simulink model "model"  (R2014a)
(part 5 of 6)

  _CN_240522248_230000_CN_261953891_230000/RConn1 -- T_261953891__/LConn1 -- _CN_261953891_230000_CN_262122922_230000/RConn1
  _CN_240522248_230000_CN_261953891_230000/RConn2 -- T_261953891__/LConn2 -- _CN_261953891_230000_CN_262122922_230000/RConn2
  _CN_240522248_230000_CN_261953891_230000/RConn3 -- T_261953891__/LConn3 -- _CN_261953891_230000_CN_262122922_230000/RConn3 -- bus92/LConn1
  T_204336141__/LConn1 -- _CN_204336141_230000_CN_194446718_230000/LConn1
  T_204336141__/LConn2 -- _CN_204336141_230000_CN_194446718_230000/LConn2
  _CN_204336141_230000_CN_194446718_230000/LConn3 -- T_204336141__/LConn3 -- bus93/LConn1
  T_194446718__Santa_Maria_3/LConn1 -- _CN_204336141_230000_CN_194446718_230000/RConn1
  T_194446718__Santa_Maria_3/LConn2 -- _CN_204336141_230000_CN_194446718_230000/RConn2
  _CN_204336141_230000_CN_194446718_230000/RConn3 -- T_194446718__Santa_Maria_3/LConn3 -- bus94/LConn1
  _CN_146723856_230000_CN_105353506_230000/LConn1 -- T_146723856_230000_Subestação_Maringá/LConn1 -- _CN_146723856_230000_CN_206109551_230000/LConn1 -- _CN_146723856_230000_CN_394083271_230000/LConn1
  _CN_146723856_230000_CN_105353506_230000/LConn2 -- T_146723856_230000_Subestação_Maringá/LConn2 -- _CN_146723856_230000_CN_206109551_230000/LConn2 -- _CN_146723856_230000_CN_394083271_230000/LConn2
  _CN_146723856_230000_CN_105353506_230000/LConn3 -- T_146723856_230000_Subestação_Maringá/LConn3 -- _CN_146723856_230000_CN_206109551_230000/LConn3 -- _CN_146723856_230000_CN_394083271_230000/LConn3 -- bus95/LConn1
  _CN_146723856_230000_CN_105353506_230000/RConn1 -- T_105353506_230000_Subestação_Apucarana/LConn1 -- Linha_de_Transmissão_CM_AP_CN_105353506_230000_CN_394083271_230000/LConn1 -- _CN_131689631_230000_CN_105353506_230000/LConn1 -- _CN_105361984_230000_CN_105353506_230000/LConn1
  _CN_146723856_230000_CN_105353506_230000/RConn2 -- T_105353506_230000_Subestação_Apucarana/LConn2 -- Linha_de_Transmissão_CM_AP_CN_105353506_230000_CN_394083271_230000/LConn2 -- _CN_131689631_230000_CN_105353506_230000/LConn2 -- _CN_105361984_230000_CN_105353506_230000/LConn2
  _CN_146723856_230000_CN_105353506_230000/RConn3 -- T_105353506_230000_Subestação_Apucarana/LConn3 -- Linha_de_Transmissão_CM_AP_CN_105353506_230000_CN_394083271_230000/LConn3 -- bus96/LConn1 -- _CN_131689631_230000_CN_105353506_230000/LConn3 -- _CN_105361984_230000_CN_105353506_230000/LConn3
  T_206109551_230000_Subestação_Sarandi/LConn1 -- _CN_146723856_230000_CN_206109551_230000/RConn1
  T_206109551_230000_Subestação_Sarandi/LConn2 -- _CN_146723856_230000_CN_206109551_230000/RConn2
  _CN_146723856_230000_CN_206109551_230000/RConn3 -- T_206109551_230000_Subestação_Sarandi/LConn3 -- bus97/LConn1
  _CN_146723856_230000_CN_394083271_230000/RConn1 -- T_394083271_230000;13800_Subestação_Campo_Mourão/LConn1 -- Linha_de_Transmissão_CM_AP_CN_105353506_230000_CN_394083271_230000/RConn1
  _CN_146723856_230000_CN_394083271_230000/RConn2 -- T_394083271_230000;13800_Subestação_Campo_Mourão/LConn2 -- Linha_de_Transmissão_CM_AP_CN_105353506_230000_CN_394083271_230000/RConn2
  _CN_146723856_230000_CN_394083271_230000/RConn3 -- T_394083271_230000;13800_Subestação_Campo_Mourão/LConn3 -- Linha_de_Transmissão_CM_AP_CN_105353506_230000_CN_394083271_230000/RConn3 -- bus98/LConn1
  _CN_323557394_230000_CN_303915320_230000/LConn1 -- T_323557394__/RConn1 -- L_323557394/LConn1
  _CN_323557394_230000_CN_303915320_230000/LConn2 -- T_323557394__/RConn2 -- L_323557394/LConn2
  _CN_323557394_230000_CN_303915320_230000/LConn3 -- T_323557394__/RConn3 -- L_323557394/LConn3 -- bus99/LConn1
  T_303915320__/LConn1 -- _CN_323557394_230000_CN_303915320_230000/RConn1
  T_303915320__/LConn2 -- _CN_323557394_230000_CN_303915320_230000/RConn2
  _CN_323557394_230000_CN_303915320_230000/RConn3 -- T_303915320__/LConn3 -- bus100/LConn1
  _CN_262826007_230000_CN_262826015_230000/LConn1 -- T_262826007__/RConn1 -- L_262826007/LConn1
  _CN_262826007_230000_CN_262826015_230000/LConn2 -- T_262826007__/RConn2 -- L_262826007/LConn2
  _CN_262826007_230000_CN_262826015_230000/LConn3 -- T_262826007__/RConn3 -- L_262826007/LConn3 -- bus101/LConn1
  T_262826015__/LConn1 -- _CN_262826007_230000_CN_262826015_230000/RConn1
  T_262826015__/LConn2 -- _CN_262826007_230000_CN_262826015_230000/RConn2
  _CN_262826007_230000_CN_262826015_230000/RConn3 -- T_262826015__/LConn3 -- bus102/LConn1
  _CN_241914909_230000_CN_241914913_230000/LConn1 -- T_241914909__/LConn1 -- _CN_241914909_230000_CN_241914935_230000/LConn1 -- _CN_241914909_230000_CN_242506367_230000/LConn1 -- _CN_241914909_230000_CN_242506209_230000/LConn1
  _CN_241914909_230000_CN_241914913_230000/LConn2 -- T_241914909__/LConn2 -- _CN_241914909_230000_CN_241914935_230000/LConn2 -- _CN_241914909_230000_CN_242506367_230000/LConn2 -- _CN_241914909_230000_CN_242506209_230000/LConn2
  _CN_241914909_230000_CN_241914913_230000/LConn3 -- T_241914909__/LConn3 -- _CN_241914909_230000_CN_241914935_230000/LConn3 -- _CN_241914909_230000_CN_242506367_230000/LConn3 -- bus103/LConn1 -- _CN_241914909_230000_CN_242506209_230000/LConn3
  _CN_241914909_230000_CN_241914913_230000/RConn1 -- T_241914913__/RConn1 -- L_241914913/LConn1
  _CN_241914909_230000_CN_241914913_230000/RConn2 -- T_241914913__/RConn2 -- L_241914913/LConn2
  _CN_241914909_230000_CN_241914913_230000/RConn3 -- T_241914913__/RConn3 -- L_241914913/LConn3 -- bus104/LConn1
  T_242506209__/LConn1 -- _CN_241914909_230000_CN_242506209_230000/RConn1
  T_242506209__/LConn2 -- _CN_241914909_230000_CN_242506209_230000/RConn2
  _CN_241914909_230000_CN_242506209_230000/RConn3 -- T_242506209__/LConn3 -- bus105/LConn1
  T_241914935__/LConn1 -- _CN_241914909_230000_CN_241914935_230000/RConn1
  T_241914935__/LConn2 -- _CN_241914909_230000_CN_241914935_230000/RConn2
  _CN_241914909_230000_CN_241914935_230000/RConn3 -- T_241914935__/LConn3 -- bus106/LConn1
  T_242506367__/LConn1 -- _CN_241914909_230000_CN_242506367_230000/RConn1
  T_242506367__/LConn2 -- _CN_241914909_230000_CN_242506367_230000/RConn2
  _CN_241914909_230000_CN_242506367_230000/RConn3 -- T_242506367__/LConn3 -- bus107/LConn1
  T_171490854__Subestação_UHE_Itiquira/LConn1 -- LT_Itiquira___Rondonópolis_CN_171490854_230000_CN_45415932_230000/LConn1
  T_171490854__Subestação_UHE_Itiquira/LConn2 -- LT_Itiquira___Rondonópolis_CN_171490854_230000_CN_45415932_230000/LConn2
  LT_Itiquira___Rondonópolis_CN_171490854_230000_CN_45415932_230000/LConn3 -- T_171490854__Subestação_UHE_Itiquira/LConn3 -- bus108/LConn1
  LT_Itiquira___Rondonópolis_CN_171490854_230000_CN_45415932_230000/RConn1 -- T_45415932__Subestação_Rondonópolis/LConn1 -- LT_Rondonópolis___Cuiabá_CN_168664395_230000_CN_45415932_230000/LConn1 -- LT_Rio_Verde___Rondonópolis_CN_174643089_230000_CN_45415932_230000/LConn1 -- LT_Rondonópolis___Coxipó_C2_CN_320803018_230000_CN_45415932_230000/LConn1 -- LT_Rio_Verde___Barra_do_Peixe___Rondonópolis_CN_260845415_230000_CN_45415932_230000/LConn1
  LT_Itiquira___Rondonópolis_CN_171490854_230000_CN_45415932_230000/RConn2 -- T_45415932__Subestação_Rondonópolis/LConn2 -- LT_Rondonópolis___Cuiabá_CN_168664395_230000_CN_45415932_230000/LConn2 -- LT_Rio_Verde___Rondonópolis_CN_174643089_230000_CN_45415932_230000/LConn2 -- LT_Rondonópolis___Coxipó_C2_CN_320803018_230000_CN_45415932_230000/LConn2 -- LT_Rio_Verde___Barra_do_Peixe___Rondonópolis_CN_260845415_230000_CN_45415932_230000/LConn2
  LT_Itiquira___Rondonópolis_CN_171490854_230000_CN_45415932_230000/RConn3 -- T_45415932__Subestação_Rondonópolis/LConn3 -- LT_Rondonópolis___Cuiabá_CN_168664395_230000_CN_45415932_230000/LConn3 -- bus109/LConn1 -- LT_Rio_Verde___Rondonópolis_CN_174643089_230000_CN_45415932_230000/LConn3 -- LT_Rondonópolis___Coxipó_C2_CN_320803018_230000_CN_45415932_230000/LConn3 -- LT_Rio_Verde___Barra_do_Peixe___Rondonópolis_CN_260845415_230000_CN_45415932_230000/LConn3
  _CN_291611826_230000_CN_291608487_230000/LConn1 -- T_291611826__Subestação_da_CELG/LConn1 -- _CN_291611826_230000_CN_306133422_230000/LConn1 -- _CN_291611826_230000_CN_142370065_230000/LConn1
  _CN_291611826_230000_CN_291608487_230000/LConn2 -- T_291611826__Subestação_da_CELG/LConn2 -- _CN_291611826_230000_CN_306133422_230000/LConn2 -- _CN_291611826_230000_CN_142370065_230000/LConn2
  _CN_291611826_230000_CN_291608487_230000/LConn3 -- T_291611826__Subestação_da_CELG/LConn3 -- _CN_291611826_230000_CN_306133422_230000/LConn3 -- _CN_291611826_230000_CN_142370065_230000/LConn3 -- bus110/LConn1
  T_291608487__/LConn1 -- _CN_291611826_230000_CN_291608487_230000/RConn1
  T_291608487__/LConn2 -- _CN_291611826_230000_CN_291608487_230000/RConn2
  _CN_291611826_230000_CN_291608487_230000/RConn3 -- T_291608487__/LConn3 -- bus111/LConn1
  _CN_291611826_230000_CN_306133422_230000/RConn1 -- T_306133422__Subestação_Anhanguera/RConn1 -- _CN_256782587_230000_CN_306133422_230000/LConn1
  _CN_291611826_230000_CN_306133422_230000/RConn2 -- T_306133422__Subestação_Anhanguera/RConn2 -- _CN_256782587_230000_CN_306133422_230000/LConn2
  _CN_291611826_230000_CN_306133422_230000/RConn3 -- T_306133422__Subestação_Anhanguera/RConn3 -- _CN_256782587_230000_CN_306133422_230000/LConn3 -- bus112/LConn1
  _CN_291611826_230000_CN_142370065_230000/RConn1 -- T_142370065__Subestação_Brasília_Sul/RConn1 -- L_142370065/LConn1
  _CN_291611826_230000_CN_142370065_230000/RConn2 -- T_142370065__Subestação_Brasília_Sul/RConn2 -- L_142370065/LConn2
  _CN_291611826_230000_CN_142370065_230000/RConn3 -- T_142370065__Subestação_Brasília_Sul/RConn3 -- L_142370065/LConn3 -- bus113/LConn1
  T_282046525__Subestação_de_energia_elétrica_de_Itaituba/LConn1 -- Tucuruí___Itaituba_CN_282046525_230000_CN_320566584_230000/LConn1
  T_282046525__Subestação_de_energia_elétrica_de_Itaituba/LConn2 -- Tucuruí___Itaituba_CN_282046525_230000_CN_320566584_230000/LConn2
  Tucuruí___Itaituba_CN_282046525_230000_CN_320566584_230000/LConn3 -- T_282046525__Subestação_de_energia_elétrica_de_Itaituba/LConn3 -- bus114/LConn1
  T_320566584__/LConn1 -- Tucuruí___Itaituba_CN_282046525_230000_CN_320566584_230000/RConn1
  T_320566584__/LConn2 -- Tucuruí___Itaituba_CN_282046525_230000_CN_320566584_230000/RConn2
  Tucuruí___Itaituba_CN_282046525_230000_CN_320566584_230000/RConn3 -- T_320566584__/LConn3 -- bus115/LConn1
  T_306908735__Subestação_Barreiras/LConn1 -- Bom_Jesus_da_Lapa___Barreiras_CN_306908735_230000_CN_320600566_230000/LConn1
  T_306908735__Subestação_Barreiras/LConn2 -- Bom_Jesus_da_Lapa___Barreiras_CN_306908735_230000_CN_320600566_230000/LConn2
  Bom_Jesus_da_Lapa___Barreiras_CN_306908735_230000_CN_320600566_230000/LConn3 -- T_306908735__Subestação_Barreiras/LConn3 -- bus116/LConn1
  Bom_Jesus_da_Lapa___Barreiras_CN_306908735_230000_CN_320600566_230000/RConn1 -- T_320600566__/LConn1 -- _CN_293729126_230000_CN_320600566_230000/LConn1 -- _CN_320709254_230000_CN_320600566_230000/LConn1
  Bom_Jesus_da_Lapa___Barreiras_CN_306908735_230000_CN_320600566_230000/RConn2 -- T_320600566__/LConn2 -- _CN_293729126_230000_CN_320600566_230000/LConn2 -- _CN_320709254_230000_CN_320600566_230000/LConn2
  Bom_Jesus_da_Lapa___Barreiras_CN_306908735_230000_CN_320600566_230000/RConn3 -- T_320600566__/LConn3 -- _CN_293729126_230000_CN_320600566_230000/LConn3 -- bus117/LConn1 -- _CN_320709254_230000_CN_320600566_230000/LConn3
  _CN_105361984_230000_CN_105353506_230000/RConn1 -- T_105361984__/LConn1 -- _CN_105361984_230000_CN_104822084_230000/LConn1
  _CN_105361984_230000_CN_105353506_230000/RConn2 -- T_105361984__/LConn2 -- _CN_105361984_230000_CN_104822084_230000/LConn2
  _CN_105361984_230000_CN_105353506_230000/RConn3 -- T_105361984__/LConn3 -- _CN_105361984_230000_CN_104822084_230000/LConn3 -- bus118/LConn1
  _CN_105361984_230000_CN_104822084_230000/RConn1 -- T_104822084__/RConn1 -- L_104822084/LConn1
  _CN_105361984_230000_CN_104822084_230000/RConn2 -- T_104822084__/RConn2 -- L_104822084/LConn2
  _CN_105361984_230000_CN_104822084_230000/RConn3 -- T_104822084__/RConn3 -- L_104822084/LConn3 -- bus119/LConn1
  _CN_199918657_230000_CN_204473485_230000/LConn1 -- T_199918657__/LConn1 -- _CN_199918657_230000_CN_200489312_230000/LConn1
  _CN_199918657_230000_CN_204473485_230000/LConn2 -- T_199918657__/LConn2 -- _CN_199918657_230000_CN_200489312_230000/LConn2
  _CN_199918657_230000_CN_204473485_230000/LConn3 -- T_199918657__/LConn3 -- _CN_199918657_230000_CN_200489312_230000/LConn3 -- bus120/LConn1
  _CN_199918657_230000_CN_204473485_230000/RConn1 -- T_204473485__/RConn1 -- L_204473485/LConn1
  _CN_199918657_230000_CN_204473485_230000/RConn2 -- T_204473485__/RConn2 -- L_204473485/LConn2
  _CN_199918657_230000_CN_204473485_230000/RConn3 -- T_204473485__/RConn3 -- L_204473485/LConn3 -- bus121/LConn1
  T_200489312__Passo_Real/LConn1 -- _CN_199918657_230000_CN_200489312_230000/RConn1
  T_200489312__Passo_Real/LConn2 -- _CN_199918657_230000_CN_200489312_230000/RConn2
  _CN_199918657_230000_CN_200489312_230000/RConn3 -- T_200489312__Passo_Real/LConn3 -- bus122/LConn1
  T_271789127__Subestação_De_Porto_Velho/LConn1 -- Porto_Velho___Abunã_CN_271789127_230000_CN_232080998_230000/LConn1
  T_271789127__Subestação_De_Porto_Velho/LConn2 -- Porto_Velho___Abunã_CN_271789127_230000_CN_232080998_230000/LConn2
  Porto_Velho___Abunã_CN_271789127_230000_CN_232080998_230000/LConn3 -- T_271789127__Subestação_De_Porto_Velho/LConn3 -- bus123/LConn1
  T_232080998__/LConn1 -- Porto_Velho___Abunã_CN_271789127_230000_CN_232080998_230000/RConn1
  T_232080998__/LConn2 -- Porto_Velho___Abunã_CN_271789127_230000_CN_232080998_230000/RConn2
  Porto_Velho___Abunã_CN_271789127_230000_CN_232080998_230000/RConn3 -- T_232080998__/LConn3 -- bus124/LConn1
  _CN_253518922_230000_CN_253296634_230000/LConn1 -- T_253518922__/LConn1 -- _CN_253518922_230000_CN_251440816_230000/LConn1
  _CN_253518922_230000_CN_253296634_230000/LConn2 -- T_253518922__/LConn2 -- _CN_253518922_230000_CN_251440816_230000/LConn2
  _CN_253518922_230000_CN_253296634_230000/LConn3 -- T_253518922__/LConn3 -- _CN_253518922_230000_CN_251440816_230000/LConn3 -- bus125/LConn1
  _CN_253518922_230000_CN_253296634_230000/RConn1 -- T_253296634__/LConn1 -- _CN_253338257_230000_CN_253296634_230000/LConn1
  _CN_253518922_230000_CN_253296634_230000/RConn2 -- T_253296634__/LConn2 -- _CN_253338257_230000_CN_253296634_230000/LConn2
  _CN_253518922_230000_CN_253296634_230000/RConn3 -- T_253296634__/LConn3 -- _CN_253338257_230000_CN_253296634_230000/LConn3 -- bus126/LConn1
  _CN_253518922_230000_CN_251440816_230000/RConn1 -- T_251440816__/LConn1 -- _CN_253509480_230000_CN_251440816_230000/LConn1 -- _CN_251440816_230000_CN_255316432_230000/LConn1
  _CN_253518922_230000_CN_251440816_230000/RConn2 -- T_251440816__/LConn2 -- _CN_253509480_230000_CN_251440816_230000/LConn2 -- _CN_251440816_230000_CN_255316432_230000/LConn2
  _CN_253518922_230000_CN_251440816_230000/RConn3 -- T_251440816__/LConn3 -- _CN_253509480_230000_CN_251440816_230000/LConn3 -- _CN_251440816_230000_CN_255316432_230000/LConn3 -- bus127/LConn1
  T_171063374__/LConn1 -- LT_Nobres___Coxipó_CN_171063374_230000_CN_320803018_230000/LConn1
  T_171063374__/LConn2 -- LT_Nobres___Coxipó_CN_171063374_230000_CN_320803018_230000/LConn2
  LT_Nobres___Coxipó_CN_171063374_230000_CN_320803018_230000/LConn3 -- T_171063374__/LConn3 -- bus128/LConn1
  LT_Nobres___Coxipó_CN_171063374_230000_CN_320803018_230000/RConn1 -- T_320803018__Subestação_Coxipó/LConn1 -- LT_Rondonópolis___Coxipó_C2_CN_320803018_230000_CN_45415932_230000/RConn1 -- LT_Cuiabá___Coxipó_CN_320803018_230000_CN_168664395_230000/LConn1 -- _CN_168904844_230000_CN_320803018_230000/LConn1
  LT_Nobres___Coxipó_CN_171063374_230000_CN_320803018_230000/RConn2 -- T_320803018__Subestação_Coxipó/LConn2 -- LT_Rondonópolis___Coxipó_C2_CN_320803018_230000_CN_45415932_230000/RConn2 -- LT_Cuiabá___Coxipó_CN_320803018_230000_CN_168664395_230000/LConn2 -- _CN_168904844_230000_CN_320803018_230000/LConn2
  LT_Nobres___Coxipó_CN_171063374_230000_CN_320803018_230000/RConn3 -- T_320803018__Subestação_Coxipó/LConn3 -- LT_Rondonópolis___Coxipó_C2_CN_320803018_230000_CN_45415932_230000/RConn3 -- LT_Cuiabá___Coxipó_CN_320803018_230000_CN_168664395_230000/LConn3 -- bus129/LConn1 -- _CN_168904844_230000_CN_320803018_230000/LConn3
  _CN_247879262_230000_CN_200004360_230000/LConn1 -- T_247879262__Subestação_Biguaçu/RConn1 -- _CN_247879262_230000_CN_25102262_230000/LConn1 -- L_247879262/LConn1
  _CN_247879262_230000_CN_200004360_230000/LConn2 -- T_247879262__Subestação_Biguaçu/RConn2 -- _CN_247879262_230000_CN_25102262_230000/LConn2 -- L_247879262/LConn2
  _CN_247879262_230000_CN_200004360_230000/LConn3 -- T_247879262__Subestação_Biguaçu/RConn3 -- _CN_247879262_230000_CN_25102262_230000/LConn3 -- L_247879262/LConn3 -- bus130/LConn1
  T_200004360__Substação_Palhoça/LConn1 -- _CN_247879262_230000_CN_200004360_230000/RConn1
  T_200004360__Substação_Palhoça/LConn2 -- _CN_247879262_230000_CN_200004360_230000/RConn2
  _CN_247879262_230000_CN_200004360_230000/RConn3 -- T_200004360__Substação_Palhoça/LConn3 -- bus131/LConn1
  _CN_247879262_230000_CN_25102262_230000/RConn1 -- T_25102262__Subestação_Blumenau/RConn1 -- _CN_421202632_230000_CN_25102262_230000/LConn1 -- L_25102262/LConn1
  _CN_247879262_230000_CN_25102262_230000/RConn2 -- T_25102262__Subestação_Blumenau/RConn2 -- _CN_421202632_230000_CN_25102262_230000/LConn2 -- L_25102262/LConn2
  _CN_247879262_230000_CN_25102262_230000/RConn3 -- T_25102262__Subestação_Blumenau/RConn3 -- _CN_421202632_230000_CN_25102262_230000/LConn3 -- L_25102262/LConn3 -- bus132/LConn1
  T_260344421__Subestação_Brasnorte/LConn1 -- LT_Brasnorte___Juína_CN_260344421_230000_CN_313073391_230000/LConn1
  T_260344421__Subestação_Brasnorte/LConn2 -- LT_Brasnorte___Juína_CN_260344421_230000_CN_313073391_230000/LConn2
  LT_Brasnorte___Juína_CN_260344421_230000_CN_313073391_230000/LConn3 -- T_260344421__Subestação_Brasnorte/LConn3 -- bus133/LConn1
  T_313073391__/LConn1 -- LT_Brasnorte___Juína_CN_260344421_230000_CN_313073391_230000/RConn1
  T_313073391__/LConn2 -- LT_Brasnorte___Juína_CN_260344421_230000_CN_313073391_230000/RConn2
  LT_Brasnorte___Juína_CN_260344421_230000_CN_313073391_230000/RConn3 -- T_313073391__/LConn3 -- bus134/LConn1
  LT_Rio_Verde___Barra_do_Peixe___Rondonópolis_CN_260845415_230000_CN_174643089_230000/LConn1 -- T_260845415__Subestação_Barra_do_Peixe/LConn1 -- LT_Rio_Verde___Barra_do_Peixe___Rondonópolis_CN_260845415_230000_CN_45415932_230000/RConn1 -- LT_Ribeirãozinho___Barra_do_Peixe_CN_260845415_230000_CN_260845416_230000/LConn1
  LT_Rio_Verde___Barra_do_Peixe___Rondonópolis_CN_260845415_230000_CN_174643089_230000/LConn2 -- T_260845415__Subestação_Barra_do_Peixe/LConn2 -- LT_Rio_Verde___Barra_do_Peixe___Rondonópolis_CN_260845415_230000_CN_45415932_230000/RConn2 -- LT_Ribeirãozinho___Barra_do_Peixe_CN_260845415_230000_CN_260845416_230000/LConn2
  LT_Rio_Verde___Barra_do_Peixe___Rondonópolis_CN_260845415_230000_CN_174643089_230000/LConn3 -- T_260845415__Subestação_Barra_do_Peixe/LConn3 -- LT_Rio_Verde___Barra_do_Peixe___Rondonópolis_CN_260845415_230000_CN_45415932_230000/RConn3 -- LT_Ribeirãozinho___Barra_do_Peixe_CN_260845415_230000_CN_260845416_230000/LConn3 -- bus135/LConn1
  LT_Rio_Verde___Barra_do_Peixe___Rondonópolis_CN_260845415_230000_CN_174643089_230000/RConn1 -- T_174643089__Rio_Verde/LConn1 -- LT_Rio_Verde___Rondonópolis_CN_174643089_230000_CN_45415932_230000/RConn1 -- LT_Itumbiara___Rio_Verde_CN_303270691_230000_CN_174643089_230000/LConn1
  LT_Rio_Verde___Barra_do_Peixe___Rondonópolis_CN_260845415_230000_CN_174643089_230000/RConn2 -- T_174643089__Rio_Verde/LConn2 -- LT_Rio_Verde___Rondonópolis_CN_174643089_230000_CN_45415932_230000/RConn2 -- LT_Itumbiara___Rio_Verde_CN_303270691_230000_CN_174643089_230000/LConn2
  LT_Rio_Verde___Barra_do_Peixe___Rondonópolis_CN_260845415_230000_CN_174643089_230000/RConn3 -- T_174643089__Rio_Verde/LConn3 -- LT_Rio_Verde___Rondonópolis_CN_174643089_230000_CN_45415932_230000/RConn3 -- bus136/LConn1 -- LT_Itumbiara___Rio_Verde_CN_303270691_230000_CN_174643089_230000/LConn3
  LT_Ribeirãozinho___Barra_do_Peixe_CN_260845415_230000_CN_260845416_230000/RConn1 -- T_260845416__Subestação_Ribeirãozinho/RConn1 -- L_260845416/LConn1
  LT_Ribeirãozinho___Barra_do_Peixe_CN_260845415_230000_CN_260845416_230000/RConn2 -- T_260845416__Subestação_Ribeirãozinho/RConn2 -- L_260845416/LConn2
  LT_Ribeirãozinho___Barra_do_Peixe_CN_260845415_230000_CN_260845416_230000/RConn3 -- T_260845416__Subestação_Ribeirãozinho/RConn3 -- L_260845416/LConn3 -- bus137/LConn1
  T_253509480__/LConn1 -- _CN_253509480_230000_CN_251440816_230000/RConn1
  T_253509480__/LConn2 -- _CN_253509480_230000_CN_251440816_230000/RConn2
  _CN_253509480_230000_CN_251440816_230000/RConn3 -- T_253509480__/LConn3 -- bus138/LConn1
  T_237588091_230000_/LConn1 -- _CN_237588091_230000_CN_237588075_230000/LConn1
  T_237588091_230000_/LConn2 -- _CN_237588091_230000_CN_237588075_230000/LConn2
  _CN_237588091_230000_CN_237588075_230000/LConn3 -- T_237588091_230000_/LConn3 -- bus139/LConn1
  G_237588075_Casa_de_Força_UHE_Mauá/RConn1 -- _CN_237588091_230000_CN_237588075_230000/RConn1
  G_237588075_Casa_de_Força_UHE_Mauá/RConn2 -- _CN_237588091_230000_CN_237588075_230000/RConn2
  _CN_237588091_230000_CN_237588075_230000/RConn3 -- G_237588075_Casa_de_Força_UHE_Mauá/RConn3 -- bus140/LConn1
  T_172447363__/LConn1 -- _CN_172447363_230000_CN_293811021_230000/LConn1
  T_172447363__/LConn2 -- _CN_172447363_230000_CN_293811021_230000/LConn2
  _CN_172447363_230000_CN_293811021_230000/LConn3 -- T_172447363__/LConn3 -- bus141/LConn1
  _CN_172447363_230000_CN_293811021_230000/RConn1 -- T_293811021__Subestação_Ibicoara/RConn1 -- L_293811021/LConn1
  _CN_172447363_230000_CN_293811021_230000/RConn2 -- T_293811021__Subestação_Ibicoara/RConn2 -- L_293811021/LConn2
  _CN_172447363_230000_CN_293811021_230000/RConn3 -- T_293811021__Subestação_Ibicoara/RConn3 -- L_293811021/LConn3 -- bus142/LConn1
  _CN_320709254_230000_CN_320600566_230000/RConn1 -- T_320709254__/LConn1 -- _CN_320709254_230000_CN_255983102_230000/LConn1
  _CN_320709254_230000_CN_320600566_230000/RConn2 -- T_320709254__/LConn2 -- _CN_320709254_230000_CN_255983102_230000/LConn2
  _CN_320709254_230000_CN_320600566_230000/RConn3 -- T_320709254__/LConn3 -- _CN_320709254_230000_CN_255983102_230000/LConn3 -- bus143/LConn1
  T_255983102__/LConn1 -- _CN_320709254_230000_CN_255983102_230000/RConn1
  T_255983102__/LConn2 -- _CN_320709254_230000_CN_255983102_230000/RConn2
  _CN_320709254_230000_CN_255983102_230000/RConn3 -- T_255983102__/LConn3 -- bus144/LConn1
  T_168904844__Subestação_Jauru/LConn1 -- _CN_168904844_230000_CN_320803018_230000/RConn1
  T_168904844__Subestação_Jauru/LConn2 -- _CN_168904844_230000_CN_320803018_230000/RConn2
  _CN_168904844_230000_CN_320803018_230000/RConn3 -- T_168904844__Subestação_Jauru/LConn3 -- bus145/LConn1
  T_253338257__/LConn1 -- _CN_253338257_230000_CN_253296634_230000/RConn1
  T_253338257__/LConn2 -- _CN_253338257_230000_CN_253296634_230000/RConn2
  _CN_253338257_230000_CN_253296634_230000/RConn3 -- T_253338257__/LConn3 -- bus146/LConn1
  T_276741266__/LConn1 -- _CN_276741266_230000_CN_161482453_230000/LConn1
  T_276741266__/LConn2 -- _CN_276741266_230000_CN_161482453_230000/LConn2
  _CN_276741266_230000_CN_161482453_230000/LConn3 -- T_276741266__/LConn3 -- bus147/LConn1
  T_161482453_230000_Subestação_Manaus/LConn1 -- _CN_276741266_230000_CN_161482453_230000/RConn1
  T_161482453_230000_Subestação_Manaus/LConn2 -- _CN_276741266_230000_CN_161482453_230000/RConn2
  _CN_276741266_230000_CN_161482453_230000/RConn3 -- T_161482453_230000_Subestação_Manaus/LConn3 -- bus148/LConn1
  T_131689631__/LConn1 -- _CN_131689631_230000_CN_105353506_230000/RConn1
  T_131689631__/LConn2 -- _CN_131689631_230000_CN_105353506_230000/RConn2
  _CN_131689631_230000_CN_105353506_230000/RConn3 -- T_131689631__/LConn3 -- bus149/LConn1
  T_150728362__/LConn1 -- _CN_150728362_230000_CN_206686474_230000/LConn1
  T_150728362__/LConn2 -- _CN_150728362_230000_CN_206686474_230000/LConn2
  _CN_150728362_230000_CN_206686474_230000/LConn3 -- T_150728362__/LConn3 -- bus150/LConn1
  _CN_150728362_230000_CN_206686474_230000/RConn1 -- T_206686474_230000;138000;13800_Subestação_Xanxerê_Eletrosul/LConn1 -- _CN_240027358_230000_CN_206686474_230000/LConn1 -- _CN_206686474_230000_CN_174067174_230000/LConn1
  _CN_150728362_230000_CN_206686474_230000/RConn2 -- T_206686474_230000;138000;13800_Subestação_Xanxerê_Eletrosul/LConn2 -- _CN_240027358_230000_CN_206686474_230000/LConn2 -- _CN_206686474_230000_CN_174067174_230000/LConn2
  _CN_150728362_230000_CN_206686474_230000/RConn3 -- T_206686474_230000;138000;13800_Subestação_Xanxerê_Eletrosul/LConn3 -- _CN_240027358_230000_CN_206686474_230000/LConn3 -- _CN_206686474_230000_CN_174067174_230000/LConn3 -- bus151/LConn1
  T_422987951__/LConn1 -- _CN_422987951_230000_CN_140181432_230000/LConn1
  T_422987951__/LConn2 -- _CN_422987951_230000_CN_140181432_230000/LConn2
  _CN_422987951_230000_CN_140181432_230000/LConn3 -- T_422987951__/LConn3 -- bus152/LConn1
  _CN_422987951_230000_CN_140181432_230000/RConn1 -- T_140181432__Subestação_Campos_Novos/RConn1 -- _CN_130128162_230000_CN_140181432_230000/LConn1 -- L_140181432/LConn1
  _CN_422987951_230000_CN_140181432_230000/RConn2 -- T_140181432__Subestação_Campos_Novos/RConn2 -- _CN_130128162_230000_CN_140181432_230000/LConn2 -- L_140181432/LConn2
  _CN_422987951_230000_CN_140181432_230000/RConn3 -- T_140181432__Subestação_Campos_Novos/RConn3 -- _CN_130128162_230000_CN_140181432_230000/LConn3 -- L_140181432/LConn3 -- bus153/LConn1
  _CN_251440816_230000_CN_255316432_230000/RConn1 -- T_255316432__Subestação_de_Barro_Alto/LConn1 -- _CN_255316432_230000_CN_255316445_230000/LConn1
  _CN_251440816_230000_CN_255316432_230000/RConn2 -- T_255316432__Subestação_de_Barro_Alto/LConn2 -- _CN_255316432_230000_CN_255316445_230000/LConn2
  _CN_251440816_230000_CN_255316432_230000/RConn3 -- T_255316432__Subestação_de_Barro_Alto/LConn3 -- _CN_255316432_230000_CN_255316445_230000/LConn3 -- bus154/LConn1
  T_421202632__Subestação_Jorge_Lacerda_B/LConn1 -- _CN_421202632_230000_CN_25102262_230000/RConn1
  T_421202632__Subestação_Jorge_Lacerda_B/LConn2 -- _CN_421202632_230000_CN_25102262_230000/RConn2
  _CN_421202632_230000_CN_25102262_230000/RConn3 -- T_421202632__Subestação_Jorge_Lacerda_B/LConn3 -- bus155/LConn1
  _CN_262608562_230000_CN_262600085_230000/RConn1 -- T_262608562__/LConn1 -- _CN_262608562_230000_CN_262659852_230000/LConn1 -- _CN_262608562_230000_CN_203819294_230000/LConn1
  _CN_262608562_230000_CN_262600085_230000/RConn2 -- T_262608562__/LConn2 -- _CN_262608562_230000_CN_262659852_230000/LConn2 -- _CN_262608562_230000_CN_203819294_230000/LConn2
  _CN_262608562_230000_CN_262600085_230000/RConn3 -- T_262608562__/LConn3 -- _CN_262608562_230000_CN_262659852_230000/LConn3 -- _CN_262608562_230000_CN_203819294_230000/LConn3 -- bus156/LConn1
  _CN_262608562_230000_CN_262659852_230000/RConn1 -- G_262659852_/RConn1 -- _CN_262608719_230000_CN_262659852_230000/LConn1
  _CN_262608562_230000_CN_262659852_230000/RConn2 -- G_262659852_/RConn2 -- _CN_262608719_230000_CN_262659852_230000/LConn2
  _CN_262608562_230000_CN_262659852_230000/RConn3 -- G_262659852_/RConn3 -- _CN_262608719_230000_CN_262659852_230000/LConn3 -- bus157/LConn1
  G_203819294_Usina_Termelétrica_Pecém/RConn1 -- _CN_262608562_230000_CN_203819294_230000/RConn1
  G_203819294_Usina_Termelétrica_Pecém/RConn2 -- _CN_262608562_230000_CN_203819294_230000/RConn2
  _CN_262608562_230000_CN_203819294_230000/RConn3 -- G_203819294_Usina_Termelétrica_Pecém/RConn3 -- bus158/LConn1
  T_204496577__/LConn1 -- _CN_204496577_230000_CN_121809567_230000/LConn1
  T_204496577__/LConn2 -- _CN_204496577_230000_CN_121809567_230000/LConn2
  _CN_204496577_230000_CN_121809567_230000/LConn3 -- T_204496577__/LConn3 -- bus159/LConn1
  _CN_204496577_230000_CN_121809567_230000/RConn1 -- T_121809567__Livramento_2/LConn1 -- _CN_221918263_230000_CN_121809567_230000/LConn1
  _CN_204496577_230000_CN_121809567_230000/RConn2 -- T_121809567__Livramento_2/LConn2 -- _CN_221918263_230000_CN_121809567_230000/LConn2
  _CN_204496577_230000_CN_121809567_230000/RConn3 -- T_121809567__Livramento_2/LConn3 -- _CN_221918263_230000_CN_121809567_230000/LConn3 -- bus160/LConn1
  _CN_196020936_230000_CN_285303568_230000/LConn1 -- T_196020936__/RConn1 -- _CN_196020936_230000_CN_271352019_230000/LConn1 -- L_196020936/LConn1
  _CN_196020936_230000_CN_285303568_230000/LConn2 -- T_196020936__/RConn2 -- _CN_196020936_230000_CN_271352019_230000/LConn2 -- L_196020936/LConn2
  _CN_196020936_230000_CN_285303568_230000/LConn3 -- T_196020936__/RConn3 -- _CN_196020936_230000_CN_271352019_230000/LConn3 -- L_196020936/LConn3 -- bus161/LConn1
  T_285303568__Subestação_de_Picos/LConn1 -- _CN_196020936_230000_CN_285303568_230000/RConn1
  T_285303568__Subestação_de_Picos/LConn2 -- _CN_196020936_230000_CN_285303568_230000/RConn2
  _CN_196020936_230000_CN_285303568_230000/RConn3 -- T_285303568__Subestação_de_Picos/LConn3 -- bus162/LConn1
  T_271352019__/LConn1 -- _CN_196020936_230000_CN_271352019_230000/RConn1
  T_271352019__/LConn2 -- _CN_196020936_230000_CN_271352019_230000/RConn2
  _CN_196020936_230000_CN_271352019_230000/RConn3 -- T_271352019__/LConn3 -- bus163/LConn1
  LT_Cuiabá___Coxipó_CN_320803018_230000_CN_168664395_230000/RConn1 -- T_168664395__Subestação_Cuiabá/RConn1 -- LT_Rondonópolis___Cuiabá_CN_168664395_230000_CN_45415932_230000/RConn1 -- L_168664395/LConn1
  LT_Cuiabá___Coxipó_CN_320803018_230000_CN_168664395_230000/RConn2 -- T_168664395__Subestação_Cuiabá/RConn2 -- LT_Rondonópolis___Cuiabá_CN_168664395_230000_CN_45415932_230000/RConn2 -- L_168664395/LConn2
  LT_Cuiabá___Coxipó_CN_320803018_230000_CN_168664395_230000/RConn3 -- T_168664395__Subestação_Cuiabá/RConn3 -- LT_Rondonópolis___Cuiabá_CN_168664395_230000_CN_45415932_230000/RConn3 -- L_168664395/LConn3 -- bus164/LConn1
  _CN_130128162_230000_CN_140181432_230000/RConn1 -- T_130128162__/LConn1 -- _CN_130128162_230000_CN_358443834_230000/LConn1
  _CN_130128162_230000_CN_140181432_230000/RConn2 -- T_130128162__/LConn2 -- _CN_130128162_230000_CN_358443834_230000/LConn2
  _CN_130128162_230000_CN_140181432_230000/RConn3 -- T_130128162__/LConn3 -- _CN_130128162_230000_CN_358443834_230000/LConn3 -- bus165/LConn1
  T_358443834__/LConn1 -- _CN_130128162_230000_CN_358443834_230000/RConn1
  T_358443834__/LConn2 -- _CN_130128162_230000_CN_358443834_230000/RConn2
  _CN_130128162_230000_CN_358443834_230000/RConn3 -- T_358443834__/LConn3 -- bus166/LConn1
  T_240027358__Subestação_UHE_Passo_Fundo/LConn1 -- _CN_240027358_230000_CN_206686474_230000/RConn1
  T_240027358__Subestação_UHE_Passo_Fundo/LConn2 -- _CN_240027358_230000_CN_206686474_230000/RConn2
  _CN_240027358_230000_CN_206686474_230000/RConn3 -- T_240027358__Subestação_UHE_Passo_Fundo/LConn3 -- bus167/LConn1
  T_251109605__Sub_estação_da_Coelba/LConn1 -- _CN_251109605_230000_CN_307509505_230000/LConn1
  T_251109605__Sub_estação_da_Coelba/LConn2 -- _CN_251109605_230000_CN_307509505_230000/LConn2
  _CN_251109605_230000_CN_307509505_230000/LConn3 -- T_251109605__Sub_estação_da_Coelba/LConn3 -- bus168/LConn1
  T_307509505__Coelba/LConn1 -- _CN_251109605_230000_CN_307509505_230000/RConn1
  T_307509505__Coelba/LConn2 -- _CN_251109605_230000_CN_307509505_230000/RConn2
  _CN_251109605_230000_CN_307509505_230000/RConn3 -- T_307509505__Coelba/LConn3 -- bus169/LConn1
  _CN_256782575_230000_CN_430982316_230000/LConn1 -- T_256782575__Cachoeira_Dourada/LConn1 -- LT_Itumbiara___Cachoeira_Dourada_CN_256782575_230000_CN_303270691_230000/LConn1 -- _CN_256782575_230000_CN_256782587_230000/LConn1
  _CN_256782575_230000_CN_430982316_230000/LConn2 -- T_256782575__Cachoeira_Dourada/LConn2 -- LT_Itumbiara___Cachoeira_Dourada_CN_256782575_230000_CN_303270691_230000/LConn2 -- _CN_256782575_230000_CN_256782587_230000/LConn2
  _CN_256782575_230000_CN_430982316_230000/LConn3 -- T_256782575__Cachoeira_Dourada/LConn3 -- LT_Itumbiara___Cachoeira_Dourada_CN_256782575_230000_CN_303270691_230000/LConn3 -- bus170/LConn1 -- _CN_256782575_230000_CN_256782587_230000/LConn3
  G_430982316_UHE_Cachoeira_Dourada/RConn1 -- _CN_256782575_230000_CN_430982316_230000/RConn1
  G_430982316_UHE_Cachoeira_Dourada/RConn2 -- _CN_256782575_230000_CN_430982316_230000/RConn2
  _CN_256782575_230000_CN_430982316_230000/RConn3 -- G_430982316_UHE_Cachoeira_Dourada/RConn3 -- bus171/LConn1
  _CN_256782575_230000_CN_256782587_230000/RConn1 -- T_256782587__/LConn1 -- _CN_256782587_230000_CN_306133422_230000/RConn1
  _CN_256782575_230000_CN_256782587_230000/RConn2 -- T_256782587__/LConn2 -- _CN_256782587_230000_CN_306133422_230000/RConn2
  _CN_256782575_230000_CN_256782587_230000/RConn3 -- T_256782587__/LConn3 -- _CN_256782587_230000_CN_306133422_230000/RConn3 -- bus172/LConn1
  LT_Itumbiara___Cachoeira_Dourada_CN_256782575_230000_CN_303270691_230000/RConn1 -- T_303270691__Subestação_da_UHE_Itumbiara/RConn1 -- LT_Itumbiara___Rio_Verde_CN_303270691_230000_CN_174643089_230000/RConn1 -- _CN_303270691_230000_CN_361594711_230000/LConn1 -- L_303270691/LConn1
  LT_Itumbiara___Cachoeira_Dourada_CN_256782575_230000_CN_303270691_230000/RConn2 -- T_303270691__Subestação_da_UHE_Itumbiara/RConn2 -- LT_Itumbiara___Rio_Verde_CN_303270691_230000_CN_174643089_230000/RConn2 -- _CN_303270691_230000_CN_361594711_230000/LConn2 -- L_303270691/LConn2
  LT_Itumbiara___Cachoeira_Dourada_CN_256782575_230000_CN_303270691_230000/RConn3 -- T_303270691__Subestação_da_UHE_Itumbiara/RConn3 -- LT_Itumbiara___Rio_Verde_CN_303270691_230000_CN_174643089_230000/RConn3 -- _CN_303270691_230000_CN_361594711_230000/LConn3 -- L_303270691/LConn3 -- bus173/LConn1
  T_194829553__Subestação_Figueira/LConn1 -- Linha_SE_Figueira_SE_Ponta_Grossa_Norte_CN_194829553_230000_CN_306588466_230000/LConn1
  T_194829553__Subestação_Figueira/LConn2 -- Linha_SE_Figueira_SE_Ponta_Grossa_Norte_CN_194829553_230000_CN_306588466_230000/LConn2
  Linha_SE_Figueira_SE_Ponta_Grossa_Norte_CN_194829553_230000_CN_306588466_230000/LConn3 -- T_194829553__Subestação_Figueira/LConn3 -- bus174/LConn1
  Linha_SE_Figueira_SE_Ponta_Grossa_Norte_CN_194829553_230000_CN_306588466_230000/RConn1 -- T_306588466__Subestação_Ponta_Grossa_Norte/LConn1 -- Linha_SE_Areia_SE_Ponta_Grossa_Norte_CN_316971776_230000_CN_306588466_230000/LConn1
  Linha_SE_Figueira_SE_Ponta_Grossa_Norte_CN_194829553_230000_CN_306588466_230000/RConn2 -- T_306588466__Subestação_Ponta_Grossa_Norte/LConn2 -- Linha_SE_Areia_SE_Ponta_Grossa_Norte_CN_316971776_230000_CN_306588466_230000/LConn2
  Linha_SE_Figueira_SE_Ponta_Grossa_Norte_CN_194829553_230000_CN_306588466_230000/RConn3 -- T_306588466__Subestação_Ponta_Grossa_Norte/LConn3 -- Linha_SE_Areia_SE_Ponta_Grossa_Norte_CN_316971776_230000_CN_306588466_230000/LConn3 -- bus175/LConn1
  _CN_316971776_230000_CN_131742617_230000/LConn1 -- T_316971776__Substação_Areia/RConn1 -- Linha_SE_Areia_SE_Ponta_Grossa_Norte_CN_316971776_230000_CN_306588466_230000/RConn1 -- L_316971776/LConn1
  _CN_316971776_230000_CN_131742617_230000/LConn2 -- T_316971776__Substação_Areia/RConn2 -- Linha_SE_Areia_SE_Ponta_Grossa_Norte_CN_316971776_230000_CN_306588466_230000/RConn2 -- L_316971776/LConn2
  _CN_316971776_230000_CN_131742617_230000/LConn3 -- T_316971776__Substação_Areia/RConn3 -- Linha_SE_Areia_SE_Ponta_Grossa_Norte_CN_316971776_230000_CN_306588466_230000/RConn3 -- L_316971776/LConn3 -- bus176/LConn1
  _CN_316971776_230000_CN_131742617_230000/RConn1 -- T_131742617__/RConn1 -- L_131742617/LConn1
  _CN_316971776_230000_CN_131742617_230000/RConn2 -- T_131742617__/RConn2 -- L_131742617/LConn2
  _CN_316971776_230000_CN_131742617_230000/RConn3 -- T_131742617__/RConn3 -- L_131742617/LConn3 -- bus177/LConn1
  T_283835652__Subestação_da_UHE_Dardanelos/LConn1 -- LT_UHE_Dardanelos___Juína_CN_283835652_230000_CN_260845425_230000/LConn1
  T_283835652__Subestação_da_UHE_Dardanelos/LConn2 -- LT_UHE_Dardanelos___Juína_CN_283835652_230000_CN_260845425_230000/LConn2
  LT_UHE_Dardanelos___Juína_CN_283835652_230000_CN_260845425_230000/LConn3 -- T_283835652__Subestação_da_UHE_Dardanelos/LConn3 -- bus178/LConn1
  LT_UHE_Dardanelos___Juína_CN_283835652_230000_CN_260845425_230000/RConn1 -- T_260845425__Subestação_Juína/LConn1 -- LT_Nova_Mutum___Brasnorte___Juína_CN_260845424_230000_CN_260845425_230000/LConn1
  LT_UHE_Dardanelos___Juína_CN_283835652_230000_CN_260845425_230000/RConn2 -- T_260845425__Subestação_Juína/LConn2 -- LT_Nova_Mutum___Brasnorte___Juína_CN_260845424_230000_CN_260845425_230000/LConn2
  LT_UHE_Dardanelos___Juína_CN_283835652_230000_CN_260845425_230000/RConn3 -- T_260845425__Subestação_Juína/LConn3 -- LT_Nova_Mutum___Brasnorte___Juína_CN_260845424_230000_CN_260845425_230000/LConn3 -- bus179/LConn1
  T_174067174_230000;135000_Subestação_Foz_do_Chapecó/LConn1 -- _CN_206686474_230000_CN_174067174_230000/RConn1
  T_174067174_230000;135000_Subestação_Foz_do_Chapecó/LConn2 -- _CN_206686474_230000_CN_174067174_230000/RConn2
  _CN_206686474_230000_CN_174067174_230000/RConn3 -- T_174067174_230000;135000_Subestação_Foz_do_Chapecó/LConn3 -- bus180/LConn1
  T_361594711__/LConn1 -- _CN_303270691_230000_CN_361594711_230000/RConn1
  T_361594711__/LConn2 -- _CN_303270691_230000_CN_361594711_230000/RConn2
  _CN_303270691_230000_CN_361594711_230000/RConn3 -- T_361594711__/LConn3 -- bus181/LConn1
  T_336967460_230000_/LConn1 -- _CN_336967460_230000_CN_336967459_230000/LConn1
  T_336967460_230000_/LConn2 -- _CN_336967460_230000_CN_336967459_230000/LConn2
  _CN_336967460_230000_CN_336967459_230000/LConn3 -- T_336967460_230000_/LConn3 -- bus182/LConn1
  T_336967459_230000_/LConn1 -- _CN_336967460_230000_CN_336967459_230000/RConn1
  T_336967459_230000_/LConn2 -- _CN_336967460_230000_CN_336967459_230000/RConn2
  _CN_336967460_230000_CN_336967459_230000/RConn3 -- T_336967459_230000_/LConn3 -- bus183/LConn1
  T_262932268__/LConn1 -- Linha_de_Transmissão_Boa_Esperança___Teresina_CN_262932268_230000_CN_263232825_230000/LConn1
  T_262932268__/LConn2 -- Linha_de_Transmissão_Boa_Esperança___Teresina_CN_262932268_230000_CN_263232825_230000/LConn2
  Linha_de_Transmissão_Boa_Esperança___Teresina_CN_262932268_230000_CN_263232825_230000/LConn3 -- T_262932268__/LConn3 -- bus184/LConn1
  Linha_de_Transmissão_Boa_Esperança___Teresina_CN_262932268_230000_CN_263232825_230000/RConn1 -- T_263232825__/RConn1 -- L_263232825/LConn1
  Linha_de_Transmissão_Boa_Esperança___Teresina_CN_262932268_230000_CN_263232825_230000/RConn2 -- T_263232825__/RConn2 -- L_263232825/LConn2
  Linha_de_Transmissão_Boa_Esperança___Teresina_CN_262932268_230000_CN_263232825_230000/RConn3 -- T_263232825__/RConn3 -- L_263232825/LConn3 -- bus185/LConn1
  T_221918263__Subestação_Coletora_Cerro_Chato/LConn1 -- _CN_221918263_230000_CN_121809567_230000/RConn1
  T_221918263__Subestação_Coletora_Cerro_Chato/LConn2 -- _CN_221918263_230000_CN_121809567_230000/RConn2
  _CN_221918263_230000_CN_121809567_230000/RConn3 -- T_221918263__Subestação_Coletora_Cerro_Chato/LConn3 -- bus186/LConn1
  T_262608719__/LConn1 -- _CN_262608719_230000_CN_262659852_230000/RConn1
  T_262608719__/LConn2 -- _CN_262608719_230000_CN_262659852_230000/RConn2
  _CN_262608719_230000_CN_262659852_230000/RConn3 -- T_262608719__/LConn3 -- bus187/LConn1
  T_216234332__/LConn1 -- _CN_216234332_230000_CN_215284729_230000/LConn1
  T_216234332__/LConn2 -- _CN_216234332_230000_CN_215284729_230000/LConn2
  _CN_216234332_230000_CN_215284729_230000/LConn3 -- T_216234332__/LConn3 -- bus188/LConn1
  _CN_216234332_230000_CN_215284729_230000/RConn1 -- T_215284729__/RConn1 -- L_215284729/LConn1
  _CN_216234332_230000_CN_215284729_230000/RConn2 -- T_215284729__/RConn2 -- L_215284729/LConn2
  _CN_216234332_230000_CN_215284729_230000/RConn3 -- T_215284729__/RConn3 -- L_215284729/LConn3 -- bus189/LConn1
  T_271227236__/LConn1 -- LT_Ribeiro_Gonçalves___Balsas_CN_271227236_230000_CN_271242661_230000/LConn1
  T_271227236__/LConn2 -- LT_Ribeiro_Gonçalves___Balsas_CN_271227236_230000_CN_271242661_230000/LConn2
  LT_Ribeiro_Gonçalves___Balsas_CN_271227236_230000_CN_271242661_230000/LConn3 -- T_271227236__/LConn3 -- bus190/LConn1
  LT_Ribeiro_Gonçalves___Balsas_CN_271227236_230000_CN_271242661_230000/RConn1 -- T_271242661__Subestação_Ribeiro_Gonçalves/RConn1 -- L_271242661/LConn1
  LT_Ribeiro_Gonçalves___Balsas_CN_271227236_230000_CN_271242661_230000/RConn2 -- T_271242661__Subestação_Ribeiro_Gonçalves/RConn2 -- L_271242661/LConn2
  LT_Ribeiro_Gonçalves___Balsas_CN_271227236_230000_CN_271242661_230000/RConn3 -- T_271242661__Subestação_Ribeiro_Gonçalves/RConn3 -- L_271242661/LConn3 -- bus191/LConn1
  _CN_293729126_230000_CN_320600566_230000/RConn1 -- T_293729126__Bom_Jesus_da_Lapa/RConn1 -- L_293729126/LConn1
  _CN_293729126_230000_CN_320600566_230000/RConn2 -- T_293729126__Bom_Jesus_da_Lapa/RConn2 -- L_293729126/LConn2
  _CN_293729126_230000_CN_320600566_230000/RConn3 -- T_293729126__Bom_Jesus_da_Lapa/RConn3 -- L_293729126/LConn3 -- bus192/LConn1
  T_41756817__Cidade_Industrial/LConn1 -- _CN_41756817_230000_CN_94745966_230000/LConn1
  T_41756817__Cidade_Industrial/LConn2 -- _CN_41756817_230000_CN_94745966_230000/LConn2
  _CN_41756817_230000_CN_94745966_230000/LConn3 -- T_41756817__Cidade_Industrial/LConn3 -- bus193/LConn1
  _CN_41756817_230000_CN_94745966_230000/RConn1 -- T_94745966__Nova_Santa_Rita/RConn1 -- L_94745966/LConn1
  _CN_41756817_230000_CN_94745966_230000/RConn2 -- T_94745966__Nova_Santa_Rita/RConn2 -- L_94745966/LConn2
  _CN_41756817_230000_CN_94745966_230000/RConn3 -- T_94745966__Nova_Santa_Rita/RConn3 -- L_94745966/LConn3 -- bus194/LConn1
  T_260845424__/LConn1 -- LT_Nova_Mutum___Brasnorte___Juína_CN_260845424_230000_CN_260845425_230000/RConn1
  T_260845424__/LConn2 -- LT_Nova_Mutum___Brasnorte___Juína_CN_260845424_230000_CN_260845425_230000/RConn2
  LT_Nova_Mutum___Brasnorte___Juína_CN_260845424_230000_CN_260845425_230000/RConn3 -- T_260845424__/LConn3 -- bus195/LConn1
  T_168946071__Subestação_Nobres/LConn1 -- LT_Nobres___Várzea_Grande_CN_168946071_230000_CN_169406381_230000/LConn1
  T_168946071__Subestação_Nobres/LConn2 -- LT_Nobres___Várzea_Grande_CN_168946071_230000_CN_169406381_230000/LConn2
  LT_Nobres___Várzea_Grande_CN_168946071_230000_CN_169406381_230000/LConn3 -- T_168946071__Subestação_Nobres/LConn3 -- bus196/LConn1
  T_169406381__Subestação_Trevo_do_Lagarto/LConn1 -- LT_Nobres___Várzea_Grande_CN_168946071_230000_CN_169406381_230000/RConn1
  T_169406381__Subestação_Trevo_do_Lagarto/LConn2 -- LT_Nobres___Várzea_Grande_CN_168946071_230000_CN_169406381_230000/RConn2
  LT_Nobres___Várzea_Grande_CN_168946071_230000_CN_169406381_230000/RConn3 -- T_169406381__Subestação_Trevo_do_Lagarto/LConn3 -- bus197/LConn1
  _CN_295701344_230000_CN_390741811_230000/LConn1 -- T_295701344__/RConn1 -- L_295701344/LConn1
  _CN_295701344_230000_CN_390741811_230000/LConn2 -- T_295701344__/RConn2 -- L_295701344/LConn2
  _CN_295701344_230000_CN_390741811_230000/LConn3 -- T_295701344__/RConn3 -- L_295701344/LConn3 -- bus198/LConn1
  G_390741811_Usina_Hidrelétrica_Luiz_Eduardo_Magalhães_(Lageado)/RConn1 -- _CN_295701344_230000_CN_390741811_230000/RConn1
  G_390741811_Usina_Hidrelétrica_Luiz_Eduardo_Magalhães_(Lageado)/RConn2 -- _CN_295701344_230000_CN_390741811_230000/RConn2
  _CN_295701344_230000_CN_390741811_230000/RConn3 -- G_390741811_Usina_Hidrelétrica_Luiz_Eduardo_Magalhães_(Lageado)/RConn3 -- bus199/LConn1
  T_255316445__/LConn1 -- _CN_255316432_230000_CN_255316445_230000/RConn1
  T_255316445__/LConn2 -- _CN_255316432_230000_CN_255316445_230000/RConn2
  _CN_255316432_230000_CN_255316445_230000/RConn3 -- T_255316445__/LConn3 -- bus200/LConn1
  T_171732982__Subestação_Sinop/LConn1 -- LT_Sorriso___Sinop_C1_CN_171732982_230000_CN_171732983_230000/RConn1
  T_171732982__Subestação_Sinop/LConn2 -- LT_Sorriso___Sinop_C1_CN_171732982_230000_CN_171732983_230000/RConn2
  LT_Sorriso___Sinop_C1_CN_171732982_230000_CN_171732983_230000/RConn3 -- T_171732982__Subestação_Sinop/LConn3 -- bus201/LConn1
  _CN_180757892_345000_CN_306133422_345000/LConn1 -- T_180757892__Subestação_Samambaia/RConn1 -- _CN_180757892_345000_CN_142370065_345000/LConn1 -- L_180757892/LConn1
  _CN_180757892_345000_CN_306133422_345000/LConn2 -- T_180757892__Subestação_Samambaia/RConn2 -- _CN_180757892_345000_CN_142370065_345000/LConn2 -- L_180757892/LConn2
  _CN_180757892_345000_CN_306133422_345000/LConn3 -- T_180757892__Subestação_Samambaia/RConn3 -- _CN_180757892_345000_CN_142370065_345000/LConn3 -- L_180757892/LConn3 -- bus202/LConn1
  _CN_180757892_345000_CN_306133422_345000/RConn1 -- T_306133422__Subestação_Anhanguera/LConn1 -- _CN_306133422_345000_CN_303270691_345000/LConn1
  _CN_180757892_345000_CN_306133422_345000/RConn2 -- T_306133422__Subestação_Anhanguera/LConn2 -- _CN_306133422_345000_CN_303270691_345000/LConn2
  _CN_180757892_345000_CN_306133422_345000/RConn3 -- T_306133422__Subestação_Anhanguera/LConn3 -- _CN_306133422_345000_CN_303270691_345000/LConn3 -- bus203/LConn1
  _CN_180757892_345000_CN_142370065_345000/RConn1 -- T_142370065__Subestação_Brasília_Sul/LConn1 -- _CN_259401772_345000_CN_142370065_345000/LConn1
  _CN_180757892_345000_CN_142370065_345000/RConn2 -- T_142370065__Subestação_Brasília_Sul/LConn2 -- _CN_259401772_345000_CN_142370065_345000/LConn2
  _CN_180757892_345000_CN_142370065_345000/RConn3 -- T_142370065__Subestação_Brasília_Sul/LConn3 -- _CN_259401772_345000_CN_142370065_345000/LConn3 -- bus204/LConn1
  _CN_259401772_345000_CN_303270691_345000/LConn1 -- T_259401772__Subestação_de_Corumbá_I/LConn1 -- _CN_259401772_345000_CN_142370065_345000/RConn1
  _CN_259401772_345000_CN_303270691_345000/LConn2 -- T_259401772__Subestação_de_Corumbá_I/LConn2 -- _CN_259401772_345000_CN_142370065_345000/RConn2
  _CN_259401772_345000_CN_303270691_345000/LConn3 -- T_259401772__Subestação_de_Corumbá_I/LConn3 -- _CN_259401772_345000_CN_142370065_345000/RConn3 -- bus205/LConn1
  _CN_259401772_345000_CN_303270691_345000/RConn1 -- T_303270691__Subestação_da_UHE_Itumbiara/LConn1 -- _CN_226477359_345000_CN_303270691_345000/LConn1 -- _CN_154975532_345000_CN_303270691_345000/LConn1 -- _CN_306133422_345000_CN_303270691_345000/RConn1
  _CN_259401772_345000_CN_303270691_345000/RConn2 -- T_303270691__Subestação_da_UHE_Itumbiara/LConn2 -- _CN_226477359_345000_CN_303270691_345000/LConn2 -- _CN_154975532_345000_CN_303270691_345000/LConn2 -- _CN_306133422_345000_CN_303270691_345000/RConn2
  _CN_259401772_345000_CN_303270691_345000/RConn3 -- T_303270691__Subestação_da_UHE_Itumbiara/LConn3 -- _CN_226477359_345000_CN_303270691_345000/LConn3 -- _CN_154975532_345000_CN_303270691_345000/LConn3 -- _CN_306133422_345000_CN_303270691_345000/RConn3 -- bus206/LConn1
  _CN_188413965_345000_CN_244288461_345000/LConn1 -- T_188413965__/LConn1 -- _CN_188413965_345000_CN_229464678_345000/LConn1 -- _CN_188413965_345000_CN_189594688_345000/LConn1 -- _CN_188413965_345000_CN_257759769_345000/LConn1 -- _CN_188413965_345000_CN_152900437_345000/LConn1 -- _CN_188413965_345000_CN_225181494_345000/LConn1
  _CN_188413965_345000_CN_244288461_345000/LConn2 -- T_188413965__/LConn2 -- _CN_188413965_345000_CN_229464678_345000/LConn2 -- _CN_188413965_345000_CN_189594688_345000/LConn2 -- _CN_188413965_345000_CN_257759769_345000/LConn2 -- _CN_188413965_345000_CN_152900437_345000/LConn2 -- _CN_188413965_345000_CN_225181494_345000/LConn2
  _CN_188413965_345000_CN_244288461_345000/LConn3 -- T_188413965__/LConn3 -- _CN_188413965_345000_CN_229464678_345000/LConn3 -- _CN_188413965_345000_CN_189594688_345000/LConn3 -- _CN_188413965_345000_CN_257759769_345000/LConn3 -- bus207/LConn1 -- _CN_188413965_345000_CN_152900437_345000/LConn3 -- _CN_188413965_345000_CN_225181494_345000/LConn3
  T_244288461_345000;230000;138000;88000;13800_Subestação_Anhangüera/LConn1 -- _CN_188413965_345000_CN_244288461_345000/RConn1
  T_244288461_345000;230000;138000;88000;13800_Subestação_Anhangüera/LConn2 -- _CN_188413965_345000_CN_244288461_345000/RConn2
  _CN_188413965_345000_CN_244288461_345000/RConn3 -- T_244288461_345000;230000;138000;88000;13800_Subestação_Anhangüera/LConn3 -- bus208/LConn1
  T_152900437__/LConn1 -- _CN_188413965_345000_CN_152900437_345000/RConn1
  T_152900437__/LConn2 -- _CN_188413965_345000_CN_152900437_345000/RConn2
  _CN_188413965_345000_CN_152900437_345000/RConn3 -- T_152900437__/LConn3 -- bus209/LConn1
  _CN_188413965_345000_CN_225181494_345000/RConn1 -- T_225181494__Subestação_Ibiúna/RConn1 -- L_225181494/LConn1
  _CN_188413965_345000_CN_225181494_345000/RConn2 -- T_225181494__Subestação_Ibiúna/RConn2 -- L_225181494/LConn2
  _CN_188413965_345000_CN_225181494_345000/RConn3 -- T_225181494__Subestação_Ibiúna/RConn3 -- L_225181494/LConn3 -- bus210/LConn1
  T_229464678__/LConn1 -- _CN_188413965_345000_CN_229464678_345000/RConn1
  T_229464678__/LConn2 -- _CN_188413965_345000_CN_229464678_345000/RConn2
  _CN_188413965_345000_CN_229464678_345000/RConn3 -- T_229464678__/LConn3 -- bus211/LConn1
  T_189594688__/LConn1 -- _CN_188413965_345000_CN_189594688_345000/RConn1
  T_189594688__/LConn2 -- _CN_188413965_345000_CN_189594688_345000/RConn2
  _CN_188413965_345000_CN_189594688_345000/RConn3 -- T_189594688__/LConn3 -- bus212/LConn1
  _CN_188413965_345000_CN_257759769_345000/RConn1 -- T_257759769__/RConn1 -- L_257759769/LConn1
  _CN_188413965_345000_CN_257759769_345000/RConn2 -- T_257759769__/RConn2 -- L_257759769/LConn2
  _CN_188413965_345000_CN_257759769_345000/RConn3 -- T_257759769__/RConn3 -- L_257759769/LConn3 -- bus213/LConn1
  T_234150638__/LConn1 -- _CN_234150638_345000_CN_169790429_345000/LConn1
  T_234150638__/LConn2 -- _CN_234150638_345000_CN_169790429_345000/LConn2
  _CN_234150638_345000_CN_169790429_345000/LConn3 -- T_234150638__/LConn3 -- bus214/LConn1
  _CN_234150638_345000_CN_169790429_345000/RConn1 -- T_169790429__Estação_elétrica/LConn1 -- _CN_252205401_345000_CN_169790429_345000/LConn1
  _CN_234150638_345000_CN_169790429_345000/RConn2 -- T_169790429__Estação_elétrica/LConn2 -- _CN_252205401_345000_CN_169790429_345000/LConn2
  _CN_234150638_345000_CN_169790429_345000/RConn3 -- T_169790429__Estação_elétrica/LConn3 -- _CN_252205401_345000_CN_169790429_345000/LConn3 -- bus215/LConn1
  _CN_217382404_345000_CN_217292707_345000/LConn1 -- T_217382404__Usina_de_Jaguara/LConn1 -- _CN_217382404_345000_CN_318426878_345000/LConn1
  _CN_217382404_345000_CN_217292707_345000/LConn2 -- T_217382404__Usina_de_Jaguara/LConn2 -- _CN_217382404_345000_CN_318426878_345000/LConn2
  _CN_217382404_345000_CN_217292707_345000/LConn3 -- T_217382404__Usina_de_Jaguara/LConn3 -- _CN_217382404_345000_CN_318426878_345000/LConn3 -- bus216/LConn1
  _CN_217382404_345000_CN_217292707_345000/RConn1 -- T_217292707__/RConn1 -- L_217292707/LConn1
  _CN_217382404_345000_CN_217292707_345000/RConn2 -- T_217292707__/RConn2 -- L_217292707/LConn2
  _CN_217382404_345000_CN_217292707_345000/RConn3 -- T_217292707__/RConn3 -- L_217292707/LConn3 -- bus217/LConn1
  _CN_217382404_345000_CN_318426878_345000/RConn1 -- T_318426878__/LConn1 -- _CN_318426878_345000_CN_220972260_345000/LConn1 -- _CN_252205401_345000_CN_318426878_345000/LConn1
  _CN_217382404_345000_CN_318426878_345000/RConn2 -- T_318426878__/LConn2 -- _CN_318426878_345000_CN_220972260_345000/LConn2 -- _CN_252205401_345000_CN_318426878_345000/LConn2
  _CN_217382404_345000_CN_318426878_345000/RConn3 -- T_318426878__/LConn3 -- _CN_318426878_345000_CN_220972260_345000/LConn3 -- bus218/LConn1 -- _CN_252205401_345000_CN_318426878_345000/LConn3
  T_226477359__/LConn1 -- _CN_226477359_345000_CN_303270691_345000/RConn1
  T_226477359__/LConn2 -- _CN_226477359_345000_CN_303270691_345000/RConn2
  _CN_226477359_345000_CN_303270691_345000/RConn3 -- T_226477359__/LConn3 -- bus219/LConn1
  _CN_154975532_345000_CN_303270691_345000/RConn1 -- T_154975532_500000_Subestação_da_UHE_Itumbiara/RConn1 -- L_154975532/LConn1
  _CN_154975532_345000_CN_303270691_345000/RConn2 -- T_154975532_500000_Subestação_da_UHE_Itumbiara/RConn2 -- L_154975532/LConn2
  _CN_154975532_345000_CN_303270691_345000/RConn3 -- T_154975532_500000_Subestação_da_UHE_Itumbiara/RConn3 -- L_154975532/LConn3 -- bus220/LConn1
  T_182621871__/LConn1 -- _CN_182621871_345000_CN_283510602_345000/LConn1
  T_182621871__/LConn2 -- _CN_182621871_345000_CN_283510602_345000/LConn2
  _CN_182621871_345000_CN_283510602_345000/LConn3 -- T_182621871__/LConn3 -- bus221/LConn1
  _CN_182621871_345000_CN_283510602_345000/RConn1 -- T_283510602__Subestação_de_São_Gotardo/RConn1 -- L_283510602/LConn1
  _CN_182621871_345000_CN_283510602_345000/RConn2 -- T_283510602__Subestação_de_São_Gotardo/RConn2 -- L_283510602/LConn2
  _CN_182621871_345000_CN_283510602_345000/RConn3 -- T_283510602__Subestação_de_São_Gotardo/RConn3 -- L_283510602/LConn3 -- bus222/LConn1
  T_132700720__/LConn1 -- _CN_132700720_345000_CN_132700730_345000/LConn1
  T_132700720__/LConn2 -- _CN_132700720_345000_CN_132700730_345000/LConn2
  _CN_132700720_345000_CN_132700730_345000/LConn3 -- T_132700720__/LConn3 -- bus223/LConn1
  _CN_132700720_345000_CN_132700730_345000/RConn1 -- T_132700730__/LConn1 -- _CN_132700730_345000_CN_132700759_345000/LConn1
  _CN_132700720_345000_CN_132700730_345000/RConn2 -- T_132700730__/LConn2 -- _CN_132700730_345000_CN_132700759_345000/LConn2
  _CN_132700720_345000_CN_132700730_345000/RConn3 -- T_132700730__/LConn3 -- _CN_132700730_345000_CN_132700759_345000/LConn3 -- bus224/LConn1
  _CN_175909703_345000_CN_219471736_345000/LConn1 -- T_175909703__/LConn1 -- _CN_175909703_345000_CN_175909709_345000/LConn1
  _CN_175909703_345000_CN_219471736_345000/LConn2 -- T_175909703__/LConn2 -- _CN_175909703_345000_CN_175909709_345000/LConn2
  _CN_175909703_345000_CN_219471736_345000/LConn3 -- T_175909703__/LConn3 -- _CN_175909703_345000_CN_175909709_345000/LConn3 -- bus225/LConn1
  _CN_175909703_345000_CN_219471736_345000/RConn1 -- T_219471736__/LConn1 -- _CN_175909709_345000_CN_219471736_345000/LConn1
  _CN_175909703_345000_CN_219471736_345000/RConn2 -- T_219471736__/LConn2 -- _CN_175909709_345000_CN_219471736_345000/LConn2
  _CN_175909703_345000_CN_219471736_345000/RConn3 -- T_219471736__/LConn3 -- _CN_175909709_345000_CN_219471736_345000/LConn3 -- bus226/LConn1
  _CN_175909703_345000_CN_175909709_345000/RConn1 -- T_175909709__/RConn1 -- _CN_175909709_345000_CN_219471736_345000/RConn1 -- L_175909709/LConn1
  _CN_175909703_345000_CN_175909709_345000/RConn2 -- T_175909709__/RConn2 -- _CN_175909709_345000_CN_219471736_345000/RConn2 -- L_175909709/LConn2
  _CN_175909703_345000_CN_175909709_345000/RConn3 -- T_175909709__/RConn3 -- _CN_175909709_345000_CN_219471736_345000/RConn3 -- L_175909709/LConn3 -- bus227/LConn1
  T_132700759__/LConn1 -- _CN_132700730_345000_CN_132700759_345000/RConn1
  T_132700759__/LConn2 -- _CN_132700730_345000_CN_132700759_345000/RConn2
  _CN_132700730_345000_CN_132700759_345000/RConn3 -- T_132700759__/LConn3 -- bus228/LConn1
  T_108198075__Subestação_Jacarepaguá/LConn1 -- _CN_108198075_345000_CN_91627969_345000/LConn1
  T_108198075__Subestação_Jacarepaguá/LConn2 -- _CN_108198075_345000_CN_91627969_345000/LConn2
  _CN_108198075_345000_CN_91627969_345000/LConn3 -- T_108198075__Subestação_Jacarepaguá/LConn3 -- bus229/LConn1
  _CN_108198075_345000_CN_91627969_345000/RConn1 -- T_91627969__Subestação_Adrianópolis/RConn1 -- _CN_168692156_345000_CN_91627969_345000/LConn1 -- L_91627969/LConn1
  _CN_108198075_345000_CN_91627969_345000/RConn2 -- T_91627969__Subestação_Adrianópolis/RConn2 -- _CN_168692156_345000_CN_91627969_345000/LConn2 -- L_91627969/LConn2
  _CN_108198075_345000_CN_91627969_345000/RConn3 -- T_91627969__Subestação_Adrianópolis/RConn3 -- _CN_168692156_345000_CN_91627969_345000/LConn3 -- L_91627969/LConn3 -- bus230/LConn1
  _CN_168692156_345000_CN_91627969_345000/RConn1 -- T_168692156__Furnas/LConn1 -- _CN_168692156_345000_CN_154269127_345000/LConn1
  _CN_168692156_345000_CN_91627969_345000/RConn2 -- T_168692156__Furnas/LConn2 -- _CN_168692156_345000_CN_154269127_345000/LConn2
  _CN_168692156_345000_CN_91627969_345000/RConn3 -- T_168692156__Furnas/LConn3 -- _CN_168692156_345000_CN_154269127_345000/LConn3 -- bus231/LConn1
  _CN_168692156_345000_CN_154269127_345000/RConn1 -- T_154269127__/LConn1 -- _CN_154269127_345000_CN_196782331_345000/LConn1
  _CN_168692156_345000_CN_154269127_345000/RConn2 -- T_154269127__/LConn2 -- _CN_154269127_345000_CN_196782331_345000/LConn2
  _CN_168692156_345000_CN_154269127_345000/RConn3 -- T_154269127__/LConn3 -- _CN_154269127_345000_CN_196782331_345000/LConn3 -- bus232/LConn1
  _CN_174918846_345000_CN_196782331_345000/LConn1 -- T_174918846__/LConn1 -- _CN_174918846_345000_CN_319354712_345000/LConn1
  _CN_174918846_345000_CN_196782331_345000/LConn2 -- T_174918846__/LConn2 -- _CN_174918846_345000_CN_319354712_345000/LConn2
  _CN_174918846_345000_CN_196782331_345000/LConn3 -- T_174918846__/LConn3 -- _CN_174918846_345000_CN_319354712_345000/LConn3 -- bus233/LConn1
  _CN_174918846_345000_CN_196782331_345000/RConn1 -- T_196782331__/LConn1 -- _CN_154269127_345000_CN_196782331_345000/RConn1
  _CN_174918846_345000_CN_196782331_345000/RConn2 -- T_196782331__/LConn2 -- _CN_154269127_345000_CN_196782331_345000/RConn2
  _CN_174918846_345000_CN_196782331_345000/RConn3 -- T_196782331__/LConn3 -- _CN_154269127_345000_CN_196782331_345000/RConn3 -- bus234/LConn1
  _CN_174918846_345000_CN_319354712_345000/RConn1 -- T_319354712__/LConn1 -- _CN_319354712_345000_CN_252205401_345000/LConn1
  _CN_174918846_345000_CN_319354712_345000/RConn2 -- T_319354712__/LConn2 -- _CN_319354712_345000_CN_252205401_345000/LConn2
  _CN_174918846_345000_CN_319354712_345000/RConn3 -- T_319354712__/LConn3 -- _CN_319354712_345000_CN_252205401_345000/LConn3 -- bus235/LConn1
  _CN_319354712_345000_CN_252205401_345000/RConn1 -- T_252205401__/LConn1 -- _CN_252205401_345000_CN_318426878_345000/RConn1 -- _CN_252205401_345000_CN_169790429_345000/RConn1
  _CN_319354712_345000_CN_252205401_345000/RConn2 -- T_252205401__/LConn2 -- _CN_252205401_345000_CN_318426878_345000/RConn2 -- _CN_252205401_345000_CN_169790429_345000/RConn2
  _CN_319354712_345000_CN_252205401_345000/RConn3 -- T_252205401__/LConn3 -- _CN_252205401_345000_CN_318426878_345000/RConn3 -- _CN_252205401_345000_CN_169790429_345000/RConn3 -- bus236/LConn1
  G_220972260_Usina_Hidrelétrica_de_Furnas/RConn1 -- _CN_318426878_345000_CN_220972260_345000/RConn1
  G_220972260_Usina_Hidrelétrica_de_Furnas/RConn2 -- _CN_318426878_345000_CN_220972260_345000/RConn2
  _CN_318426878_345000_CN_220972260_345000/RConn3 -- G_220972260_Usina_Hidrelétrica_de_Furnas/RConn3 -- bus237/LConn1
  _CN_197950082_440000_CN_32800322_440000/LConn1 -- T_197950082__/LConn1 -- _CN_197950082_440000_CN_157028016_440000/LConn1 -- _CN_197950082_440000_CN_143581084_440000/LConn1
  _CN_197950082_440000_CN_32800322_440000/LConn2 -- T_197950082__/LConn2 -- _CN_197950082_440000_CN_157028016_440000/LConn2 -- _CN_197950082_440000_CN_143581084_440000/LConn2
  _CN_197950082_440000_CN_32800322_440000/LConn3 -- T_197950082__/LConn3 -- _CN_197950082_440000_CN_157028016_440000/LConn3 -- _CN_197950082_440000_CN_143581084_440000/LConn3 -- bus238/LConn1
  G_32800322_Usina_Hidrelétrica_Engenheiro_Sérgio_Motta/RConn1 -- _CN_197950082_440000_CN_32800322_440000/RConn1
  G_32800322_Usina_Hidrelétrica_Engenheiro_Sérgio_Motta/RConn2 -- _CN_197950082_440000_CN_32800322_440000/RConn2
  _CN_197950082_440000_CN_32800322_440000/RConn3 -- G_32800322_Usina_Hidrelétrica_Engenheiro_Sérgio_Motta/RConn3 -- bus239/LConn1
  _CN_197950082_440000_CN_157028016_440000/RConn1 -- T_157028016__/RConn1 -- _CN_157028016_440000_CN_183163485_440000/LConn1 -- L_157028016/LConn1
  _CN_197950082_440000_CN_157028016_440000/RConn2 -- T_157028016__/RConn2 -- _CN_157028016_440000_CN_183163485_440000/LConn2 -- L_157028016/LConn2
  _CN_197950082_440000_CN_157028016_440000/RConn3 -- T_157028016__/RConn3 -- _CN_157028016_440000_CN_183163485_440000/LConn3 -- L_157028016/LConn3 -- bus240/LConn1
  _CN_197950082_440000_CN_143581084_440000/RConn1 -- G_143581084_UHE_Jupiá_Engenheiro_Souza_Dias/RConn1 -- _CN_167339557_440000_CN_143581084_440000/LConn1 -- _CN_302901044_440000_CN_143581084_440000/LConn1
  _CN_197950082_440000_CN_143581084_440000/RConn2 -- G_143581084_UHE_Jupiá_Engenheiro_Souza_Dias/RConn2 -- _CN_167339557_440000_CN_143581084_440000/LConn2 -- _CN_302901044_440000_CN_143581084_440000/LConn2
  _CN_197950082_440000_CN_143581084_440000/RConn3 -- G_143581084_UHE_Jupiá_Engenheiro_Souza_Dias/RConn3 -- _CN_167339557_440000_CN_143581084_440000/LConn3 -- _CN_302901044_440000_CN_143581084_440000/LConn3 -- bus241/LConn1
  T_172071437__/LConn1 -- _CN_172071437_440000_CN_160888682_440000/LConn1
  T_172071437__/LConn2 -- _CN_172071437_440000_CN_160888682_440000/LConn2
  _CN_172071437_440000_CN_160888682_440000/LConn3 -- T_172071437__/LConn3 -- bus242/LConn1
  _CN_172071437_440000_CN_160888682_440000/RConn1 -- T_160888682__/LConn1 -- _CN_171525061_440000_CN_160888682_440000/LConn1 -- _CN_174852067_440000_CN_160888682_440000/LConn1
  _CN_172071437_440000_CN_160888682_440000/RConn2 -- T_160888682__/LConn2 -- _CN_171525061_440000_CN_160888682_440000/LConn2 -- _CN_174852067_440000_CN_160888682_440000/LConn2
  _CN_172071437_440000_CN_160888682_440000/RConn3 -- T_160888682__/LConn3 -- _CN_171525061_440000_CN_160888682_440000/LConn3 -- _CN_174852067_440000_CN_160888682_440000/LConn3 -- bus243/LConn1
  _CN_175929233_440000_CN_218090562_440000/LConn1 -- T_175929233__Subestação_de_Santo_Ângelo/LConn1 -- _CN_175929233_440000_CN_171525061_440000/LConn1 -- _CN_175929233_440000_CN_244245455_440000/LConn1 -- _CN_175929233_440000_CN_341042754_440000/LConn1
  _CN_175929233_440000_CN_218090562_440000/LConn2 -- T_175929233__Subestação_de_Santo_Ângelo/LConn2 -- _CN_175929233_440000_CN_171525061_440000/LConn2 -- _CN_175929233_440000_CN_244245455_440000/LConn2 -- _CN_175929233_440000_CN_341042754_440000/LConn2
  _CN_175929233_440000_CN_218090562_440000/LConn3 -- T_175929233__Subestação_de_Santo_Ângelo/LConn3 -- _CN_175929233_440000_CN_171525061_440000/LConn3 -- _CN_175929233_440000_CN_244245455_440000/LConn3 -- _CN_175929233_440000_CN_341042754_440000/LConn3 -- bus244/LConn1
  _CN_175929233_440000_CN_218090562_440000/RConn1 -- T_218090562__Subestação_de_Energia_Elétrica_Cteep/LConn1 -- _CN_218090562_440000_CN_186982606_440000/LConn1
  _CN_175929233_440000_CN_218090562_440000/RConn2 -- T_218090562__Subestação_de_Energia_Elétrica_Cteep/LConn2 -- _CN_218090562_440000_CN_186982606_440000/LConn2
  _CN_175929233_440000_CN_218090562_440000/RConn3 -- T_218090562__Subestação_de_Energia_Elétrica_Cteep/LConn3 -- _CN_218090562_440000_CN_186982606_440000/LConn3 -- bus245/LConn1
  _CN_175929233_440000_CN_171525061_440000/RConn1 -- T_171525061__Subestação/LConn1 -- _CN_167339557_440000_CN_171525061_440000/LConn1 -- _CN_302735025_440000_CN_171525061_440000/LConn1 -- _CN_171525061_440000_CN_160888682_440000/RConn1 -- LT_Água_Vermelha___Araraquara_CN_171525061_440000_CN_302931307_440000/LConn1 -- _CN_171525061_440000_CN_183163485_440000/LConn1
  _CN_175929233_440000_CN_171525061_440000/RConn2 -- T_171525061__Subestação/LConn2 -- _CN_167339557_440000_CN_171525061_440000/LConn2 -- _CN_302735025_440000_CN_171525061_440000/LConn2 -- _CN_171525061_440000_CN_160888682_440000/RConn2 -- LT_Água_Vermelha___Araraquara_CN_171525061_440000_CN_302931307_440000/LConn2 -- _CN_171525061_440000_CN_183163485_440000/LConn2
  _CN_175929233_440000_CN_171525061_440000/RConn3 -- T_171525061__Subestação/LConn3 -- _CN_167339557_440000_CN_171525061_440000/LConn3 -- _CN_302735025_440000_CN_171525061_440000/LConn3 -- _CN_171525061_440000_CN_160888682_440000/RConn3 -- LT_Água_Vermelha___Araraquara_CN_171525061_440000_CN_302931307_440000/LConn3 -- _CN_171525061_440000_CN_183163485_440000/LConn3 -- bus246/LConn1
  _CN_175929233_440000_CN_244245455_440000/RConn1 -- T_244245455__/LConn1 -- _CN_244245455_440000_CN_183163485_440000/LConn1 -- _CN_186982606_440000_CN_244245455_440000/LConn1
  _CN_175929233_440000_CN_244245455_440000/RConn2 -- T_244245455__/LConn2 -- _CN_244245455_440000_CN_183163485_440000/LConn2 -- _CN_186982606_440000_CN_244245455_440000/LConn2
  _CN_175929233_440000_CN_244245455_440000/RConn3 -- T_244245455__/LConn3 -- _CN_244245455_440000_CN_183163485_440000/LConn3 -- bus247/LConn1 -- _CN_186982606_440000_CN_244245455_440000/LConn3
  T_341042754__CESP/LConn1 -- _CN_175929233_440000_CN_341042754_440000/RConn1
  T_341042754__CESP/LConn2 -- _CN_175929233_440000_CN_341042754_440000/RConn2
  _CN_175929233_440000_CN_341042754_440000/RConn3 -- T_341042754__CESP/LConn3 -- bus248/LConn1
  _CN_157028016_440000_CN_183163485_440000/RConn1 -- T_183163485__/LConn1 -- _CN_244245455_440000_CN_183163485_440000/RConn1 -- _CN_174017677_440000_CN_183163485_440000/LConn1 -- _CN_156042539_440000_CN_183163485_440000/LConn1 -- _CN_171525061_440000_CN_183163485_440000/RConn1 -- _CN_167339557_440000_CN_183163485_440000/LConn1
  _CN_157028016_440000_CN_183163485_440000/RConn2 -- T_183163485__/LConn2 -- _CN_244245455_440000_CN_183163485_440000/RConn2 -- _CN_174017677_440000_CN_183163485_440000/LConn2 -- _CN_156042539_440000_CN_183163485_440000/LConn2 -- _CN_171525061_440000_CN_183163485_440000/RConn2 -- _CN_167339557_440000_CN_183163485_440000/LConn2
  _CN_157028016_440000_CN_183163485_440000/RConn3 -- T_183163485__/LConn3 -- _CN_244245455_440000_CN_183163485_440000/RConn3 -- bus249/LConn1 -- _CN_174017677_440000_CN_183163485_440000/LConn3 -- _CN_156042539_440000_CN_183163485_440000/LConn3 -- _CN_171525061_440000_CN_183163485_440000/RConn3 -- _CN_167339557_440000_CN_183163485_440000/LConn3
  _CN_167339557_440000_CN_286006777_440000/LConn1 -- T_167339557__/LConn1 -- _CN_167339557_440000_CN_171525061_440000/RConn1 -- _CN_167339557_440000_CN_302931307_440000/LConn1 -- _CN_167339557_440000_CN_183163485_440000/RConn1 -- _CN_167339557_440000_CN_143581084_440000/RConn1 -- _CN_167339557_440000_CN_172691560_440000/LConn1
  _CN_167339557_440000_CN_286006777_440000/LConn2 -- T_167339557__/LConn2 -- _CN_167339557_440000_CN_171525061_440000/RConn2 -- _CN_167339557_440000_CN_302931307_440000/LConn2 -- _CN_167339557_440000_CN_183163485_440000/RConn2 -- _CN_167339557_440000_CN_143581084_440000/RConn2 -- _CN_167339557_440000_CN_172691560_440000/LConn2
  _CN_167339557_440000_CN_286006777_440000/LConn3 -- T_167339557__/LConn3 -- _CN_167339557_440000_CN_171525061_440000/RConn3 -- bus250/LConn1 -- _CN_167339557_440000_CN_302931307_440000/LConn3 -- _CN_167339557_440000_CN_183163485_440000/RConn3 -- _CN_167339557_440000_CN_143581084_440000/RConn3 -- _CN_167339557_440000_CN_172691560_440000/LConn3
  _CN_167339557_440000_CN_286006777_440000/RConn1 -- T_286006777_440000_/LConn1 -- _CN_286007002_440000_CN_286006777_440000/LConn1
  _CN_167339557_440000_CN_286006777_440000/RConn2 -- T_286006777_440000_/LConn2 -- _CN_286007002_440000_CN_286006777_440000/LConn2
  _CN_167339557_440000_CN_286006777_440000/RConn3 -- T_286006777_440000_/LConn3 -- _CN_286007002_440000_CN_286006777_440000/LConn3 -- bus251/LConn1
  _CN_167339557_440000_CN_302931307_440000/RConn1 -- T_302931307_440000_LT_Água_Vermelha/RConn1 -- LT_Água_Vermelha___Araraquara_CN_171525061_440000_CN_302931307_440000/RConn1 -- _CN_174852067_440000_CN_302931307_440000/LConn1 -- L_302931307/LConn1
  _CN_167339557_440000_CN_302931307_440000/RConn2 -- T_302931307_440000_LT_Água_Vermelha/RConn2 -- LT_Água_Vermelha___Araraquara_CN_171525061_440000_CN_302931307_440000/RConn2 -- _CN_174852067_440000_CN_302931307_440000/LConn2 -- L_302931307/LConn2
  _CN_167339557_440000_CN_302931307_440000/RConn3 -- T_302931307_440000_LT_Água_Vermelha/RConn3 -- LT_Água_Vermelha___Araraquara_CN_171525061_440000_CN_302931307_440000/RConn3 -- _CN_174852067_440000_CN_302931307_440000/LConn3 -- L_302931307/LConn3 -- bus252/LConn1
  T_172691560__/LConn1 -- _CN_167339557_440000_CN_172691560_440000/RConn1
  T_172691560__/LConn2 -- _CN_167339557_440000_CN_172691560_440000/RConn2
  _CN_167339557_440000_CN_172691560_440000/RConn3 -- T_172691560__/LConn3 -- bus253/LConn1
  T_156042539__/LConn1 -- _CN_156042539_440000_CN_183163485_440000/RConn1
  T_156042539__/LConn2 -- _CN_156042539_440000_CN_183163485_440000/RConn2
  _CN_156042539_440000_CN_183163485_440000/RConn3 -- T_156042539__/LConn3 -- bus254/LConn1
  T_296110000__/LConn1 -- _CN_296110000_440000_CN_286007002_440000/LConn1
  T_296110000__/LConn2 -- _CN_296110000_440000_CN_286007002_440000/LConn2
  _CN_296110000_440000_CN_286007002_440000/LConn3 -- T_296110000__/LConn3 -- bus255/LConn1
  _CN_296110000_440000_CN_286007002_440000/RConn1 -- T_286007002_440000_/LConn1 -- _CN_286007002_440000_CN_286006777_440000/RConn1
  _CN_296110000_440000_CN_286007002_440000/RConn2 -- T_286007002_440000_/LConn2 -- _CN_286007002_440000_CN_286006777_440000/RConn2
  _CN_296110000_440000_CN_286007002_440000/RConn3 -- T_286007002_440000_/LConn3 -- _CN_286007002_440000_CN_286006777_440000/RConn3 -- bus256/LConn1
  T_302735025_440000_/LConn1 -- _CN_302735025_440000_CN_171525061_440000/RConn1
  T_302735025_440000_/LConn2 -- _CN_302735025_440000_CN_171525061_440000/RConn2
  _CN_302735025_440000_CN_171525061_440000/RConn3 -- T_302735025_440000_/LConn3 -- bus257/LConn1
  _CN_302901044_440000_CN_174017677_440000/LConn1 -- T_302901044__/LConn1 -- _CN_302901044_440000_CN_143581084_440000/RConn1
  _CN_302901044_440000_CN_174017677_440000/LConn2 -- T_302901044__/LConn2 -- _CN_302901044_440000_CN_143581084_440000/RConn2
  _CN_302901044_440000_CN_174017677_440000/LConn3 -- T_302901044__/LConn3 -- _CN_302901044_440000_CN_143581084_440000/RConn3 -- bus258/LConn1
  _CN_302901044_440000_CN_174017677_440000/RConn1 -- T_174017677_440000_/LConn1 -- _CN_174017677_440000_CN_183163485_440000/RConn1
  _CN_302901044_440000_CN_174017677_440000/RConn2 -- T_174017677_440000_/LConn2 -- _CN_174017677_440000_CN_183163485_440000/RConn2
  _CN_302901044_440000_CN_174017677_440000/RConn3 -- T_174017677_440000_/LConn3 -- _CN_174017677_440000_CN_183163485_440000/RConn3 -- bus259/LConn1
  _CN_218090562_440000_CN_186982606_440000/RConn1 -- T_186982606__/LConn1 -- _CN_186982606_440000_CN_244245455_440000/RConn1
  _CN_218090562_440000_CN_186982606_440000/RConn2 -- T_186982606__/LConn2 -- _CN_186982606_440000_CN_244245455_440000/RConn2
  _CN_218090562_440000_CN_186982606_440000/RConn3 -- T_186982606__/LConn3 -- _CN_186982606_440000_CN_244245455_440000/RConn3 -- bus260/LConn1
  _CN_174852067_440000_CN_160888682_440000/RConn1 -- T_174852067__/RConn1 -- _CN_174852067_440000_CN_302931307_440000/RConn1 -- L_174852067/LConn1
  _CN_174852067_440000_CN_160888682_440000/RConn2 -- T_174852067__/RConn2 -- _CN_174852067_440000_CN_302931307_440000/RConn2 -- L_174852067/LConn2
  _CN_174852067_440000_CN_160888682_440000/RConn3 -- T_174852067__/RConn3 -- _CN_174852067_440000_CN_302931307_440000/RConn3 -- L_174852067/LConn3 -- bus261/LConn1
  _CN_323557393_500000_CN_271191830_500000/LConn1 -- T_323557393__/LConn1 -- _CN_323557393_500000_CN_249499770_500000/LConn1 -- _CN_323557393_500000_CN_304139576_500000/LConn1
  _CN_323557393_500000_CN_271191830_500000/LConn2 -- T_323557393__/LConn2 -- _CN_323557393_500000_CN_249499770_500000/LConn2 -- _CN_323557393_500000_CN_304139576_500000/LConn2
  _CN_323557393_500000_CN_271191830_500000/LConn3 -- T_323557393__/LConn3 -- _CN_323557393_500000_CN_249499770_500000/LConn3 -- bus262/LConn1 -- _CN_323557393_500000_CN_304139576_500000/LConn3
  _CN_323557393_500000_CN_271191830_500000/RConn1 -- T_271191830__Subestação_Colinas/LConn1 -- Colinas_Sobradinho_CN_271191830_500000_CN_271242661_500000/LConn1 -- _CN_271191830_500000_CN_198634993_500000/LConn1
  _CN_323557393_500000_CN_271191830_500000/RConn2 -- T_271191830__Subestação_Colinas/LConn2 -- Colinas_Sobradinho_CN_271191830_500000_CN_271242661_500000/LConn2 -- _CN_271191830_500000_CN_198634993_500000/LConn2
  _CN_323557393_500000_CN_271191830_500000/RConn3 -- T_271191830__Subestação_Colinas/LConn3 -- Colinas_Sobradinho_CN_271191830_500000_CN_271242661_500000/LConn3 -- bus263/LConn1 -- _CN_271191830_500000_CN_198634993_500000/LConn3
  _CN_323557393_500000_CN_304139576_500000/RConn1 -- T_304139576__/LConn1 -- _CN_304139576_500000_CN_304144597_500000/LConn1
  _CN_323557393_500000_CN_304139576_500000/RConn2 -- T_304139576__/LConn2 -- _CN_304139576_500000_CN_304144597_500000/LConn2
  _CN_323557393_500000_CN_304139576_500000/RConn3 -- T_304139576__/LConn3 -- _CN_304139576_500000_CN_304144597_500000/LConn3 -- bus264/LConn1
  _CN_323557393_500000_CN_249499770_500000/RConn1 -- T_249499770__/LConn1 -- _CN_262913646_500000_CN_249499770_500000/LConn1 -- _CN_249499770_500000_CN_263232825_500000/LConn1
  _CN_323557393_500000_CN_249499770_500000/RConn2 -- T_249499770__/LConn2 -- _CN_262913646_500000_CN_249499770_500000/LConn2 -- _CN_249499770_500000_CN_263232825_500000/LConn2
  _CN_323557393_500000_CN_249499770_500000/RConn3 -- T_249499770__/LConn3 -- _CN_262913646_500000_CN_249499770_500000/LConn3 -- _CN_249499770_500000_CN_263232825_500000/LConn3 -- bus265/LConn1
  _CN_323557394_500000_CN_271524307_500000/LConn1 -- T_323557394__/LConn1 -- _CN_323557394_500000_CN_176499706_500000/LConn1
  _CN_323557394_500000_CN_271524307_500000/LConn2 -- T_323557394__/LConn2 -- _CN_323557394_500000_CN_176499706_500000/LConn2
  _CN_323557394_500000_CN_271524307_500000/LConn3 -- T_323557394__/LConn3 -- _CN_323557394_500000_CN_176499706_500000/LConn3 -- bus266/LConn1
  _CN_323557394_500000_CN_271524307_500000/RConn1 -- T_271524307__Subestação_da_Eletronorte_em_Marabá/LConn1 -- _CN_304658726_500000_CN_271524307_500000/LConn1
  _CN_323557394_500000_CN_271524307_500000/RConn2 -- T_271524307__Subestação_da_Eletronorte_em_Marabá/LConn2 -- _CN_304658726_500000_CN_271524307_500000/LConn2
  _CN_323557394_500000_CN_271524307_500000/RConn3 -- T_271524307__Subestação_da_Eletronorte_em_Marabá/LConn3 -- _CN_304658726_500000_CN_271524307_500000/LConn3 -- bus267/LConn1
  T_176499706__Açailândia/LConn1 -- _CN_323557394_500000_CN_176499706_500000/RConn1
  T_176499706__Açailândia/LConn2 -- _CN_323557394_500000_CN_176499706_500000/RConn2
  _CN_323557394_500000_CN_176499706_500000/RConn3 -- T_176499706__Açailândia/LConn3 -- bus268/LConn1
  _CN_262826007_500000_CN_262600085_500000/LConn1 -- T_262826007__/LConn1 -- _CN_262826007_500000_CN_262913646_500000/LConn1
  _CN_262826007_500000_CN_262600085_500000/LConn2 -- T_262826007__/LConn2 -- _CN_262826007_500000_CN_262913646_500000/LConn2
  _CN_262826007_500000_CN_262600085_500000/LConn3 -- T_262826007__/LConn3 -- _CN_262826007_500000_CN_262913646_500000/LConn3 -- bus269/LConn1
  _CN_262826007_500000_CN_262600085_500000/RConn1 -- T_262600085__/LConn1 -- 230kV_Chesf_CN_262559849_500000_CN_262600085_500000/LConn1
  _CN_262826007_500000_CN_262600085_500000/RConn2 -- T_262600085__/LConn2 -- 230kV_Chesf_CN_262559849_500000_CN_262600085_500000/LConn2
  _CN_262826007_500000_CN_262600085_500000/RConn3 -- T_262600085__/LConn3 -- 230kV_Chesf_CN_262559849_500000_CN_262600085_500000/LConn3 -- bus270/LConn1
  _CN_262826007_500000_CN_262913646_500000/RConn1 -- T_262913646__/LConn1 -- _CN_262913646_500000_CN_249499770_500000/RConn1
  _CN_262826007_500000_CN_262913646_500000/RConn2 -- T_262913646__/LConn2 -- _CN_262913646_500000_CN_249499770_500000/RConn2
  _CN_262826007_500000_CN_262913646_500000/RConn3 -- T_262913646__/LConn3 -- _CN_262913646_500000_CN_249499770_500000/RConn3 -- bus271/LConn1
  _CN_257759769_500000_CN_225181494_500000/LConn1 -- T_257759769__/LConn1 -- _CN_257759769_500000_CN_171525050_500000/LConn1
  _CN_257759769_500000_CN_225181494_500000/LConn2 -- T_257759769__/LConn2 -- _CN_257759769_500000_CN_171525050_500000/LConn2
  _CN_257759769_500000_CN_225181494_500000/LConn3 -- T_257759769__/LConn3 -- _CN_257759769_500000_CN_171525050_500000/LConn3 -- bus272/LConn1
  T_225181494__Subestação_Ibiúna/LConn1 -- _CN_257759769_500000_CN_225181494_500000/RConn1
  T_225181494__Subestação_Ibiúna/LConn2 -- _CN_257759769_500000_CN_225181494_500000/RConn2
  _CN_257759769_500000_CN_225181494_500000/RConn3 -- T_225181494__Subestação_Ibiúna/LConn3 -- bus273/LConn1
  _CN_257759769_500000_CN_171525050_500000/RConn1 -- T_171525050__/LConn1 -- _CN_129484075_500000_CN_171525050_500000/LConn1 -- _CN_157028016_500000_CN_171525050_500000/LConn1
  _CN_257759769_500000_CN_171525050_500000/RConn2 -- T_171525050__/LConn2 -- _CN_129484075_500000_CN_171525050_500000/LConn2 -- _CN_157028016_500000_CN_171525050_500000/LConn2
  _CN_257759769_500000_CN_171525050_500000/RConn3 -- T_171525050__/LConn3 -- _CN_129484075_500000_CN_171525050_500000/LConn3 -- bus274/LConn1 -- _CN_157028016_500000_CN_171525050_500000/LConn3
  _CN_167516187_500000_CN_131742617_500000/LConn1 -- T_167516187__Subestação_Batéias/LConn1 -- _CN_167516187_500000_CN_316971776_500000/LConn1
  _CN_167516187_500000_CN_131742617_500000/LConn2 -- T_167516187__Subestação_Batéias/LConn2 -- _CN_167516187_500000_CN_316971776_500000/LConn2
  _CN_167516187_500000_CN_131742617_500000/LConn3 -- T_167516187__Subestação_Batéias/LConn3 -- _CN_167516187_500000_CN_316971776_500000/LConn3 -- bus275/LConn1
  _CN_167516187_500000_CN_131742617_500000/RConn1 -- T_131742617__/LConn1 -- _CN_316971776_500000_CN_131742617_500000/LConn1 -- _CN_131742617_500000_CN_25102262_500000/LConn1
  _CN_167516187_500000_CN_131742617_500000/RConn2 -- T_131742617__/LConn2 -- _CN_316971776_500000_CN_131742617_500000/LConn2 -- _CN_131742617_500000_CN_25102262_500000/LConn2
  _CN_167516187_500000_CN_131742617_500000/RConn3 -- T_131742617__/LConn3 -- _CN_316971776_500000_CN_131742617_500000/LConn3 -- _CN_131742617_500000_CN_25102262_500000/LConn3 -- bus276/LConn1
  _CN_167516187_500000_CN_316971776_500000/RConn1 -- T_316971776__Substação_Areia/LConn1 -- _CN_316971776_500000_CN_131742617_500000/RConn1 -- Linha_SE_Areia_SE_Segredo_CN_150728359_500000_CN_316971776_500000/LConn1 -- _CN_316971776_500000_CN_151624015_500000/LConn1 -- _CN_316971776_500000_CN_125761911_500000/LConn1 -- _CN_316971776_500000_CN_140181432_500000/LConn1
  _CN_167516187_500000_CN_316971776_500000/RConn2 -- T_316971776__Substação_Areia/LConn2 -- _CN_316971776_500000_CN_131742617_500000/RConn2 -- Linha_SE_Areia_SE_Segredo_CN_150728359_500000_CN_316971776_500000/LConn2 -- _CN_316971776_500000_CN_151624015_500000/LConn2 -- _CN_316971776_500000_CN_125761911_500000/LConn2 -- _CN_316971776_500000_CN_140181432_500000/LConn2
  _CN_167516187_500000_CN_316971776_500000/RConn3 -- T_316971776__Substação_Areia/LConn3 -- _CN_316971776_500000_CN_131742617_500000/RConn3 -- bus277/LConn1 -- Linha_SE_Areia_SE_Segredo_CN_150728359_500000_CN_316971776_500000/LConn3 -- _CN_316971776_500000_CN_151624015_500000/LConn3 -- _CN_316971776_500000_CN_125761911_500000/LConn3 -- _CN_316971776_500000_CN_140181432_500000/LConn3
  T_241914913__/LConn1 -- LT_São_Simão___Itaguaçú_CN_241914913_500000_CN_154030807_500000/LConn1
  T_241914913__/LConn2 -- LT_São_Simão___Itaguaçú_CN_241914913_500000_CN_154030807_500000/LConn2
  LT_São_Simão___Itaguaçú_CN_241914913_500000_CN_154030807_500000/LConn3 -- T_241914913__/LConn3 -- bus278/LConn1
  LT_São_Simão___Itaguaçú_CN_241914913_500000_CN_154030807_500000/RConn1 -- T_154030807__/LConn1 -- LT_São_Simão___Jaguara_CN_154030807_500000_CN_217292707_500000/LConn1 -- _CN_154030807_500000_CN_154975532_500000/LConn1 -- _CN_154030807_500000_CN_390650772_500000/LConn1 -- _CN_154030807_500000_CN_302931307_500000/LConn1
  LT_São_Simão___Itaguaçú_CN_241914913_500000_CN_154030807_500000/RConn2 -- T_154030807__/LConn2 -- LT_São_Simão___Jaguara_CN_154030807_500000_CN_217292707_500000/LConn2 -- _CN_154030807_500000_CN_154975532_500000/LConn2 -- _CN_154030807_500000_CN_390650772_500000/LConn2 -- _CN_154030807_500000_CN_302931307_500000/LConn2
  LT_São_Simão___Itaguaçú_CN_241914913_500000_CN_154030807_500000/RConn3 -- T_154030807__/LConn3 -- LT_São_Simão___Jaguara_CN_154030807_500000_CN_217292707_500000/LConn3 -- _CN_154030807_500000_CN_154975532_500000/LConn3 -- _CN_154030807_500000_CN_390650772_500000/LConn3 -- bus279/LConn1 -- _CN_154030807_500000_CN_302931307_500000/LConn3
  LT_Itumbiara___Rio_Verde_Norte_CN_229733923_500000_CN_154975532_500000/LConn1 -- T_229733923__Subestação_Rio_Verde_Norte/LConn1 -- LT_Ribeirãozinho___Rio_Verde_CN_229733923_500000_CN_260845416_500000/LConn1
  LT_Itumbiara___Rio_Verde_Norte_CN_229733923_500000_CN_154975532_500000/LConn2 -- T_229733923__Subestação_Rio_Verde_Norte/LConn2 -- LT_Ribeirãozinho___Rio_Verde_CN_229733923_500000_CN_260845416_500000/LConn2
  LT_Itumbiara___Rio_Verde_Norte_CN_229733923_500000_CN_154975532_500000/LConn3 -- T_229733923__Subestação_Rio_Verde_Norte/LConn3 -- LT_Ribeirãozinho___Rio_Verde_CN_229733923_500000_CN_260845416_500000/LConn3 -- bus280/LConn1
  LT_Itumbiara___Rio_Verde_Norte_CN_229733923_500000_CN_154975532_500000/RConn1 -- T_154975532_500000_Subestação_da_UHE_Itumbiara/LConn1 -- _CN_154975532_500000_CN_283488616_500000/LConn1 -- _CN_154975532_500000_CN_390650772_500000/LConn1 -- _CN_154975532_500000_CN_180757892_500000/LConn1 -- _CN_154030807_500000_CN_154975532_500000/RConn1
  LT_Itumbiara___Rio_Verde_Norte_CN_229733923_500000_CN_154975532_500000/RConn2 -- T_154975532_500000_Subestação_da_UHE_Itumbiara/LConn2 -- _CN_154975532_500000_CN_283488616_500000/LConn2 -- _CN_154975532_500000_CN_390650772_500000/LConn2 -- _CN_154975532_500000_CN_180757892_500000/LConn2 -- _CN_154030807_500000_CN_154975532_500000/RConn2
  LT_Itumbiara___Rio_Verde_Norte_CN_229733923_500000_CN_154975532_500000/RConn3 -- T_154975532_500000_Subestação_da_UHE_Itumbiara/LConn3 -- _CN_154975532_500000_CN_283488616_500000/LConn3 -- _CN_154975532_500000_CN_390650772_500000/LConn3 -- _CN_154975532_500000_CN_180757892_500000/LConn3 -- bus281/LConn1 -- _CN_154030807_500000_CN_154975532_500000/RConn3
  LT_Ribeirãozinho___Rio_Verde_CN_229733923_500000_CN_260845416_500000/RConn1 -- T_260845416__Subestação_Ribeirãozinho/LConn1 -- _CN_260845416_500000_CN_168664395_500000/LConn1
  LT_Ribeirãozinho___Rio_Verde_CN_229733923_500000_CN_260845416_500000/RConn2 -- T_260845416__Subestação_Ribeirãozinho/LConn2 -- _CN_260845416_500000_CN_168664395_500000/LConn2
  LT_Ribeirãozinho___Rio_Verde_CN_229733923_500000_CN_260845416_500000/RConn3 -- T_260845416__Subestação_Ribeirãozinho/LConn3 -- _CN_260845416_500000_CN_168664395_500000/LConn3 -- bus282/LConn1
  _CN_228748856_500000_CN_247684836_500000/LConn1 -- T_228748856__Gravataí/LConn1 -- _CN_228748856_500000_CN_94745966_500000/LConn1
  _CN_228748856_500000_CN_247684836_500000/LConn2 -- T_228748856__Gravataí/LConn2 -- _CN_228748856_500000_CN_94745966_500000/LConn2
  _CN_228748856_500000_CN_247684836_500000/LConn3 -- T_228748856__Gravataí/LConn3 -- _CN_228748856_500000_CN_94745966_500000/LConn3 -- bus283/LConn1
  _CN_228748856_500000_CN_247684836_500000/RConn1 -- T_247684836__/LConn1 -- _CN_188465343_500000_CN_247684836_500000/LConn1 -- _CN_247684836_500000_CN_140181432_500000/LConn1
  _CN_228748856_500000_CN_247684836_500000/RConn2 -- T_247684836__/LConn2 -- _CN_188465343_500000_CN_247684836_500000/LConn2 -- _CN_247684836_500000_CN_140181432_500000/LConn2
  _CN_228748856_500000_CN_247684836_500000/RConn3 -- T_247684836__/LConn3 -- _CN_188465343_500000_CN_247684836_500000/LConn3 -- _CN_247684836_500000_CN_140181432_500000/LConn3 -- bus284/LConn1
  _CN_228748856_500000_CN_94745966_500000/RConn1 -- T_94745966__Nova_Santa_Rita/LConn1 -- _CN_188465343_500000_CN_94745966_500000/LConn1 -- _CN_94745966_500000_CN_140181432_500000/LConn1
  _CN_228748856_500000_CN_94745966_500000/RConn2 -- T_94745966__Nova_Santa_Rita/LConn2 -- _CN_188465343_500000_CN_94745966_500000/LConn2 -- _CN_94745966_500000_CN_140181432_500000/LConn2
  _CN_228748856_500000_CN_94745966_500000/RConn3 -- T_94745966__Nova_Santa_Rita/LConn3 -- _CN_188465343_500000_CN_94745966_500000/LConn3 -- _CN_94745966_500000_CN_140181432_500000/LConn3 -- bus285/LConn1
  T_252169283__Subestação_Vespasiano_2/LConn1 -- _CN_252169283_500000_CN_252169286_500000/LConn1
  T_252169283__Subestação_Vespasiano_2/LConn2 -- _CN_252169283_500000_CN_252169286_500000/LConn2
  _CN_252169283_500000_CN_252169286_500000/LConn3 -- T_252169283__Subestação_Vespasiano_2/LConn3 -- bus286/LConn1
  _CN_252169283_500000_CN_252169286_500000/RConn1 -- T_252169286__Subestação_Neves_1/LConn1 -- _CN_252169286_500000_CN_297523069_500000/LConn1
  _CN_252169283_500000_CN_252169286_500000/RConn2 -- T_252169286__Subestação_Neves_1/LConn2 -- _CN_252169286_500000_CN_297523069_500000/LConn2
  _CN_252169283_500000_CN_252169286_500000/RConn3 -- T_252169286__Subestação_Neves_1/LConn3 -- _CN_252169286_500000_CN_297523069_500000/LConn3 -- bus287/LConn1
  _CN_252169286_500000_CN_297523069_500000/RConn1 -- T_297523069__Sub_Estação_da_CEMIG___Bom_Despacho/LConn1 -- _CN_283510602_500000_CN_297523069_500000/LConn1
  _CN_252169286_500000_CN_297523069_500000/RConn2 -- T_297523069__Sub_Estação_da_CEMIG___Bom_Despacho/LConn2 -- _CN_283510602_500000_CN_297523069_500000/LConn2
  _CN_252169286_500000_CN_297523069_500000/RConn3 -- T_297523069__Sub_Estação_da_CEMIG___Bom_Despacho/LConn3 -- _CN_283510602_500000_CN_297523069_500000/LConn3 -- bus288/LConn1
  _CN_247879262_500000_CN_25102262_500000/LConn1 -- T_247879262__Subestação_Biguaçu/LConn1 -- _CN_247879262_500000_CN_140181432_500000/LConn1
  _CN_247879262_500000_CN_25102262_500000/LConn2 -- T_247879262__Subestação_Biguaçu/LConn2 -- _CN_247879262_500000_CN_140181432_500000/LConn2
  _CN_247879262_500000_CN_25102262_500000/LConn3 -- T_247879262__Subestação_Biguaçu/LConn3 -- _CN_247879262_500000_CN_140181432_500000/LConn3 -- bus289/LConn1
  _CN_247879262_500000_CN_25102262_500000/RConn1 -- T_25102262__Subestação_Blumenau/LConn1 -- _CN_131742617_500000_CN_25102262_500000/RConn1 -- _CN_25102262_500000_CN_140181432_500000/LConn1
  _CN_247879262_500000_CN_25102262_500000/RConn2 -- T_25102262__Subestação_Blumenau/LConn2 -- _CN_131742617_500000_CN_25102262_500000/RConn2 -- _CN_25102262_500000_CN_140181432_500000/LConn2
  _CN_247879262_500000_CN_25102262_500000/RConn3 -- T_25102262__Subestação_Blumenau/LConn3 -- _CN_131742617_500000_CN_25102262_500000/RConn3 -- _CN_25102262_500000_CN_140181432_500000/LConn3 -- bus290/LConn1
  _CN_247879262_500000_CN_140181432_500000/RConn1 -- T_140181432__Subestação_Campos_Novos/LConn1 -- _CN_25102262_500000_CN_140181432_500000/RConn1 -- _CN_188465343_500000_CN_140181432_500000/LConn1 -- _CN_247684836_500000_CN_140181432_500000/RConn1 -- _CN_316971776_500000_CN_140181432_500000/RConn1 -- _CN_94745966_500000_CN_140181432_500000/RConn1
  _CN_247879262_500000_CN_140181432_500000/RConn2 -- T_140181432__Subestação_Campos_Novos/LConn2 -- _CN_25102262_500000_CN_140181432_500000/RConn2 -- _CN_188465343_500000_CN_140181432_500000/LConn2 -- _CN_247684836_500000_CN_140181432_500000/RConn2 -- _CN_316971776_500000_CN_140181432_500000/RConn2 -- _CN_94745966_500000_CN_140181432_500000/RConn2
  _CN_247879262_500000_CN_140181432_500000/RConn3 -- T_140181432__Subestação_Campos_Novos/LConn3 -- _CN_25102262_500000_CN_140181432_500000/RConn3 -- bus291/LConn1 -- _CN_188465343_500000_CN_140181432_500000/LConn3 -- _CN_247684836_500000_CN_140181432_500000/RConn3 -- _CN_316971776_500000_CN_140181432_500000/RConn3 -- _CN_94745966_500000_CN_140181432_500000/RConn3
  _CN_253440615_500000_CN_253030804_500000/LConn1 -- T_253440615__/LConn1 -- _CN_253440615_500000_CN_253441434_500000/LConn1 -- _CN_253440615_500000_CN_253692682_500000/LConn1
  _CN_253440615_500000_CN_253030804_500000/LConn2 -- T_253440615__/LConn2 -- _CN_253440615_500000_CN_253441434_500000/LConn2 -- _CN_253440615_500000_CN_253692682_500000/LConn2
  _CN_253440615_500000_CN_253030804_500000/LConn3 -- T_253440615__/LConn3 -- _CN_253440615_500000_CN_253441434_500000/LConn3 -- _CN_253440615_500000_CN_253692682_500000/LConn3 -- bus292/LConn1
  _CN_253440615_500000_CN_253030804_500000/RConn1 -- T_253030804__Serra_da_Mesa/LConn1 -- _CN_253523129_500000_CN_253030804_500000/LConn1 -- _CN_253030804_500000_CN_259425260_500000/LConn1 -- Serra_da_Mesa___Rio_das_Éguas_CN_320600714_500000_CN_253030804_500000/LConn1
  _CN_253440615_500000_CN_253030804_500000/RConn2 -- T_253030804__Serra_da_Mesa/LConn2 -- _CN_253523129_500000_CN_253030804_500000/LConn2 -- _CN_253030804_500000_CN_259425260_500000/LConn2 -- Serra_da_Mesa___Rio_das_Éguas_CN_320600714_500000_CN_253030804_500000/LConn2
  _CN_253440615_500000_CN_253030804_500000/RConn3 -- T_253030804__Serra_da_Mesa/LConn3 -- _CN_253523129_500000_CN_253030804_500000/LConn3 -- _CN_253030804_500000_CN_259425260_500000/LConn3 -- bus293/LConn1 -- Serra_da_Mesa___Rio_das_Éguas_CN_320600714_500000_CN_253030804_500000/LConn3
  T_253441434__/LConn1 -- _CN_253440615_500000_CN_253441434_500000/RConn1
  T_253441434__/LConn2 -- _CN_253440615_500000_CN_253441434_500000/RConn2
  _CN_253440615_500000_CN_253441434_500000/RConn3 -- T_253441434__/LConn3 -- bus294/LConn1
  _CN_253440615_500000_CN_253692682_500000/RConn1 -- T_253692682__/LConn1 -- _CN_253523129_500000_CN_253692682_500000/LConn1 -- C3_CN_253692682_500000_CN_198634993_500000/LConn1
  _CN_253440615_500000_CN_253692682_500000/RConn2 -- T_253692682__/LConn2 -- _CN_253523129_500000_CN_253692682_500000/LConn2 -- C3_CN_253692682_500000_CN_198634993_500000/LConn2
  _CN_253440615_500000_CN_253692682_500000/RConn3 -- T_253692682__/LConn3 -- _CN_253523129_500000_CN_253692682_500000/LConn3 -- C3_CN_253692682_500000_CN_198634993_500000/LConn3 -- bus295/LConn1
  _CN_262559849_500000_CN_174572759_500000/LConn1 -- T_262559849__/LConn1 -- 230kV_Chesf_CN_262559849_500000_CN_262600085_500000/RConn1
  _CN_262559849_500000_CN_174572759_500000/LConn2 -- T_262559849__/LConn2 -- 230kV_Chesf_CN_262559849_500000_CN_262600085_500000/RConn2
  _CN_262559849_500000_CN_174572759_500000/LConn3 -- T_262559849__/LConn3 -- 230kV_Chesf_CN_262559849_500000_CN_262600085_500000/RConn3 -- bus296/LConn1
  _CN_262559849_500000_CN_174572759_500000/RConn1 -- T_174572759__Subestação_Milagres/LConn1 -- _CN_174572759_500000_CN_390650768_500000/LConn1
  _CN_262559849_500000_CN_174572759_500000/RConn2 -- T_174572759__Subestação_Milagres/LConn2 -- _CN_174572759_500000_CN_390650768_500000/LConn2
  _CN_262559849_500000_CN_174572759_500000/RConn3 -- T_174572759__Subestação_Milagres/LConn3 -- _CN_174572759_500000_CN_390650768_500000/LConn3 -- bus297/LConn1
  T_168664395__Subestação_Cuiabá/LConn1 -- _CN_260845416_500000_CN_168664395_500000/RConn1
  T_168664395__Subestação_Cuiabá/LConn2 -- _CN_260845416_500000_CN_168664395_500000/RConn2
  _CN_260845416_500000_CN_168664395_500000/RConn3 -- T_168664395__Subestação_Cuiabá/LConn3 -- bus298/LConn1
  _CN_249499770_500000_CN_263232825_500000/RConn1 -- T_263232825__/LConn1 -- _CN_196020936_500000_CN_263232825_500000/LConn1
  _CN_249499770_500000_CN_263232825_500000/RConn2 -- T_263232825__/LConn2 -- _CN_196020936_500000_CN_263232825_500000/LConn2
  _CN_249499770_500000_CN_263232825_500000/RConn3 -- T_263232825__/LConn3 -- _CN_196020936_500000_CN_263232825_500000/LConn3 -- bus299/LConn1
  _CN_244422281_500000_CN_158099916_500000/LConn1 -- T_244422281__Paracatu_4/LConn1 -- _CN_244422281_500000_CN_259229502_500000/LConn1 -- _CN_244422281_500000_CN_259425260_500000/LConn1 -- _CN_244422281_500000_CN_283488616_500000/LConn1
  _CN_244422281_500000_CN_158099916_500000/LConn2 -- T_244422281__Paracatu_4/LConn2 -- _CN_244422281_500000_CN_259229502_500000/LConn2 -- _CN_244422281_500000_CN_259425260_500000/LConn2 -- _CN_244422281_500000_CN_283488616_500000/LConn2
  _CN_244422281_500000_CN_158099916_500000/LConn3 -- T_244422281__Paracatu_4/LConn3 -- _CN_244422281_500000_CN_259229502_500000/LConn3 -- _CN_244422281_500000_CN_259425260_500000/LConn3 -- bus300/LConn1 -- _CN_244422281_500000_CN_283488616_500000/LConn3
  T_158099916__Pirapora_2/LConn1 -- _CN_244422281_500000_CN_158099916_500000/RConn1
  T_158099916__Pirapora_2/LConn2 -- _CN_244422281_500000_CN_158099916_500000/RConn2
  _CN_244422281_500000_CN_158099916_500000/RConn3 -- T_158099916__Pirapora_2/LConn3 -- bus301/LConn1
  _CN_244422281_500000_CN_283488616_500000/RConn1 -- T_283488616__Subestação_de_Emborcação/LConn1 -- Emborcação___São_Gotardo_CN_283510602_500000_CN_283488616_500000/LConn1 -- _CN_283488616_500000_CN_180757892_500000/LConn1 -- _CN_283488616_500000_CN_295766704_500000/LConn1 -- _CN_154975532_500000_CN_283488616_500000/RConn1
  _CN_244422281_500000_CN_283488616_500000/RConn2 -- T_283488616__Subestação_de_Emborcação/LConn2 -- Emborcação___São_Gotardo_CN_283510602_500000_CN_283488616_500000/LConn2 -- _CN_283488616_500000_CN_180757892_500000/LConn2 -- _CN_283488616_500000_CN_295766704_500000/LConn2 -- _CN_154975532_500000_CN_283488616_500000/RConn2
  _CN_244422281_500000_CN_283488616_500000/RConn3 -- T_283488616__Subestação_de_Emborcação/LConn3 -- Emborcação___São_Gotardo_CN_283510602_500000_CN_283488616_500000/LConn3 -- _CN_283488616_500000_CN_180757892_500000/LConn3 -- _CN_283488616_500000_CN_295766704_500000/LConn3 -- bus302/LConn1 -- _CN_154975532_500000_CN_283488616_500000/RConn3
  T_259229502__/LConn1 -- _CN_244422281_500000_CN_259229502_500000/RConn1
  T_259229502__/LConn2 -- _CN_244422281_500000_CN_259229502_500000/RConn2
  _CN_244422281_500000_CN_259229502_500000/RConn3 -- T_259229502__/LConn3 -- bus303/LConn1
  _CN_244422281_500000_CN_259425260_500000/RConn1 -- T_259425260__/LConn1 -- _CN_180757892_500000_CN_259425260_500000/LConn1 -- _CN_253030804_500000_CN_259425260_500000/RConn1
  _CN_244422281_500000_CN_259425260_500000/RConn2 -- T_259425260__/LConn2 -- _CN_180757892_500000_CN_259425260_500000/LConn2 -- _CN_253030804_500000_CN_259425260_500000/RConn2
  _CN_244422281_500000_CN_259425260_500000/RConn3 -- T_259425260__/LConn3 -- _CN_180757892_500000_CN_259425260_500000/LConn3 -- _CN_253030804_500000_CN_259425260_500000/RConn3 -- bus304/LConn1
  Serra_da_Mesa___Rio_das_Éguas_CN_320600714_500000_CN_253030804_500000/RConn1 -- T_320600714__Subestação_Rio_das_Éguas/LConn1 -- Rio_das_Éguas___Bom_Jesus_da_Lapa_CN_320600714_500000_CN_293729126_500000/LConn1
  Serra_da_Mesa___Rio_das_Éguas_CN_320600714_500000_CN_253030804_500000/RConn2 -- T_320600714__Subestação_Rio_das_Éguas/LConn2 -- Rio_das_Éguas___Bom_Jesus_da_Lapa_CN_320600714_500000_CN_293729126_500000/LConn2
  Serra_da_Mesa___Rio_das_Éguas_CN_320600714_500000_CN_253030804_500000/RConn3 -- T_320600714__Subestação_Rio_das_Éguas/LConn3 -- Rio_das_Éguas___Bom_Jesus_da_Lapa_CN_320600714_500000_CN_293729126_500000/LConn3 -- bus305/LConn1
  Rio_das_Éguas___Bom_Jesus_da_Lapa_CN_320600714_500000_CN_293729126_500000/RConn1 -- T_293729126__Bom_Jesus_da_Lapa/LConn1 -- Linha_de_Transmissão_Norte___Nordeste_CN_293811021_500000_CN_293729126_500000/LConn1
  Rio_das_Éguas___Bom_Jesus_da_Lapa_CN_320600714_500000_CN_293729126_500000/RConn2 -- T_293729126__Bom_Jesus_da_Lapa/LConn2 -- Linha_de_Transmissão_Norte___Nordeste_CN_293811021_500000_CN_293729126_500000/LConn2
  Rio_das_Éguas___Bom_Jesus_da_Lapa_CN_320600714_500000_CN_293729126_500000/RConn3 -- T_293729126__Bom_Jesus_da_Lapa/LConn3 -- Linha_de_Transmissão_Norte___Nordeste_CN_293811021_500000_CN_293729126_500000/LConn3 -- bus306/LConn1
  _CN_204473485_500000_CN_188465343_500000/LConn1 -- T_204473485__/LConn1 -- _CN_204473485_500000_CN_204484095_500000/LConn1
  _CN_204473485_500000_CN_188465343_500000/LConn2 -- T_204473485__/LConn2 -- _CN_204473485_500000_CN_204484095_500000/LConn2
  _CN_204473485_500000_CN_188465343_500000/LConn3 -- T_204473485__/LConn3 -- _CN_204473485_500000_CN_204484095_500000/LConn3 -- bus307/LConn1
  _CN_204473485_500000_CN_188465343_500000/RConn1 -- T_188465343__/LConn1 -- _CN_188465343_500000_CN_140181432_500000/RConn1 -- _CN_150728360_500000_CN_188465343_500000/LConn1 -- _CN_188465343_500000_CN_204484095_500000/LConn1 -- _CN_188465343_500000_CN_94745966_500000/RConn1 -- _CN_188465343_500000_CN_247684836_500000/RConn1
  _CN_204473485_500000_CN_188465343_500000/RConn2 -- T_188465343__/LConn2 -- _CN_188465343_500000_CN_140181432_500000/RConn2 -- _CN_150728360_500000_CN_188465343_500000/LConn2 -- _CN_188465343_500000_CN_204484095_500000/LConn2 -- _CN_188465343_500000_CN_94745966_500000/RConn2 -- _CN_188465343_500000_CN_247684836_500000/RConn2
  _CN_204473485_500000_CN_188465343_500000/RConn3 -- T_188465343__/LConn3 -- _CN_188465343_500000_CN_140181432_500000/RConn3 -- bus308/LConn1 -- _CN_150728360_500000_CN_188465343_500000/LConn3 -- _CN_188465343_500000_CN_204484095_500000/LConn3 -- _CN_188465343_500000_CN_94745966_500000/RConn3 -- _CN_188465343_500000_CN_247684836_500000/RConn3
  _CN_204473485_500000_CN_204484095_500000/RConn1 -- T_204484095__/LConn1 -- _CN_188465343_500000_CN_204484095_500000/RConn1
  _CN_204473485_500000_CN_204484095_500000/RConn2 -- T_204484095__/LConn2 -- _CN_188465343_500000_CN_204484095_500000/RConn2
  _CN_204473485_500000_CN_204484095_500000/RConn3 -- T_204484095__/LConn3 -- _CN_188465343_500000_CN_204484095_500000/RConn3 -- bus309/LConn1
  T_142588064__Hidroelétrica_de_Sobradinho/LConn1 -- _CN_142588064_500000_CN_390650768_500000/LConn1
  T_142588064__Hidroelétrica_de_Sobradinho/LConn2 -- _CN_142588064_500000_CN_390650768_500000/LConn2
  _CN_142588064_500000_CN_390650768_500000/LConn3 -- T_142588064__Hidroelétrica_de_Sobradinho/LConn3 -- bus310/LConn1
  _CN_142588064_500000_CN_390650768_500000/RConn1 -- T_390650768__/LConn1 -- _CN_174572759_500000_CN_390650768_500000/RConn1 -- _CN_247537019_500000_CN_390650768_500000/LConn1
  _CN_142588064_500000_CN_390650768_500000/RConn2 -- T_390650768__/LConn2 -- _CN_174572759_500000_CN_390650768_500000/RConn2 -- _CN_247537019_500000_CN_390650768_500000/LConn2
  _CN_142588064_500000_CN_390650768_500000/RConn3 -- T_390650768__/LConn3 -- _CN_174572759_500000_CN_390650768_500000/RConn3 -- _CN_247537019_500000_CN_390650768_500000/LConn3 -- bus311/LConn1
  Linha_SE_Areia_SE_Segredo_CN_150728359_500000_CN_316971776_500000/RConn1 -- T_150728359__Subestação_Segredo/LConn1 -- Linha_Segredo_Salto_Santiago_CN_150728359_500000_CN_150728360_500000/LConn1
  Linha_SE_Areia_SE_Segredo_CN_150728359_500000_CN_316971776_500000/RConn2 -- T_150728359__Subestação_Segredo/LConn2 -- Linha_Segredo_Salto_Santiago_CN_150728359_500000_CN_150728360_500000/LConn2
  Linha_SE_Areia_SE_Segredo_CN_150728359_500000_CN_316971776_500000/RConn3 -- T_150728359__Subestação_Segredo/LConn3 -- Linha_Segredo_Salto_Santiago_CN_150728359_500000_CN_150728360_500000/LConn3 -- bus312/LConn1
  Linha_Segredo_Salto_Santiago_CN_150728359_500000_CN_150728360_500000/RConn1 -- T_150728360__/LConn1 -- _CN_150728360_500000_CN_204662229_500000/LConn1 -- _CN_150728360_500000_CN_188465343_500000/RConn1 -- _CN_150728360_500000_CN_125761911_500000/LConn1
  Linha_Segredo_Salto_Santiago_CN_150728359_500000_CN_150728360_500000/RConn2 -- T_150728360__/LConn2 -- _CN_150728360_500000_CN_204662229_500000/LConn2 -- _CN_150728360_500000_CN_188465343_500000/RConn2 -- _CN_150728360_500000_CN_125761911_500000/LConn2
  Linha_Segredo_Salto_Santiago_CN_150728359_500000_CN_150728360_500000/RConn3 -- T_150728360__/LConn3 -- _CN_150728360_500000_CN_204662229_500000/LConn3 -- bus313/LConn1 -- _CN_150728360_500000_CN_188465343_500000/RConn3 -- _CN_150728360_500000_CN_125761911_500000/LConn3
  _CN_150728360_500000_CN_125761911_500000/RConn1 -- T_125761911__/LConn1 -- _CN_316971776_500000_CN_125761911_500000/RConn1 -- _CN_104822084_500000_CN_125761911_500000/LConn1 -- _CN_125761911_500000_CN_125761912_500000/LConn1 -- _CN_125761911_500000_CN_204662229_500000/LConn1
  _CN_150728360_500000_CN_125761911_500000/RConn2 -- T_125761911__/LConn2 -- _CN_316971776_500000_CN_125761911_500000/RConn2 -- _CN_104822084_500000_CN_125761911_500000/LConn2 -- _CN_125761911_500000_CN_125761912_500000/LConn2 -- _CN_125761911_500000_CN_204662229_500000/LConn2
  _CN_150728360_500000_CN_125761911_500000/RConn3 -- T_125761911__/LConn3 -- _CN_316971776_500000_CN_125761911_500000/RConn3 -- _CN_104822084_500000_CN_125761911_500000/LConn3 -- _CN_125761911_500000_CN_125761912_500000/LConn3 -- _CN_125761911_500000_CN_204662229_500000/LConn3 -- bus314/LConn1
  _CN_150728360_500000_CN_204662229_500000/RConn1 -- T_204662229__/LConn1 -- _CN_125761911_500000_CN_204662229_500000/RConn1
  _CN_150728360_500000_CN_204662229_500000/RConn2 -- T_204662229__/LConn2 -- _CN_125761911_500000_CN_204662229_500000/RConn2
  _CN_150728360_500000_CN_204662229_500000/RConn3 -- T_204662229__/LConn3 -- _CN_125761911_500000_CN_204662229_500000/RConn3 -- bus315/LConn1
  _CN_157028016_500000_CN_171525050_500000/RConn1 -- T_157028016__/LConn1 -- _CN_157028016_500000_CN_104822084_500000/LConn1
  _CN_157028016_500000_CN_171525050_500000/RConn2 -- T_157028016__/LConn2 -- _CN_157028016_500000_CN_104822084_500000/LConn2
  _CN_157028016_500000_CN_171525050_500000/RConn3 -- T_157028016__/LConn3 -- _CN_157028016_500000_CN_104822084_500000/LConn3 -- bus316/LConn1
  _CN_157028016_500000_CN_104822084_500000/RConn1 -- T_104822084__/LConn1 -- _CN_104822084_500000_CN_125761911_500000/RConn1
  _CN_157028016_500000_CN_104822084_500000/RConn2 -- T_104822084__/LConn2 -- _CN_104822084_500000_CN_125761911_500000/RConn2
  _CN_157028016_500000_CN_104822084_500000/RConn3 -- T_104822084__/LConn3 -- _CN_104822084_500000_CN_125761911_500000/RConn3 -- bus317/LConn1
  _CN_253523129_500000_CN_180757892_500000/LConn1 -- T_253523129__Subestação_UHE_Serra_da_Mesa/LConn1 -- _CN_253523129_500000_CN_253030804_500000/RConn1 -- _CN_253523129_500000_CN_253692682_500000/RConn1
  _CN_253523129_500000_CN_180757892_500000/LConn2 -- T_253523129__Subestação_UHE_Serra_da_Mesa/LConn2 -- _CN_253523129_500000_CN_253030804_500000/RConn2 -- _CN_253523129_500000_CN_253692682_500000/RConn2
  _CN_253523129_500000_CN_180757892_500000/LConn3 -- T_253523129__Subestação_UHE_Serra_da_Mesa/LConn3 -- _CN_253523129_500000_CN_253030804_500000/RConn3 -- _CN_253523129_500000_CN_253692682_500000/RConn3 -- bus318/LConn1
  _CN_253523129_500000_CN_180757892_500000/RConn1 -- T_180757892__Subestação_Samambaia/LConn1 -- _CN_154975532_500000_CN_180757892_500000/RConn1 -- _CN_283488616_500000_CN_180757892_500000/RConn1 -- _CN_180757892_500000_CN_259425260_500000/RConn1
  _CN_253523129_500000_CN_180757892_500000/RConn2 -- T_180757892__Subestação_Samambaia/LConn2 -- _CN_154975532_500000_CN_180757892_500000/RConn2 -- _CN_283488616_500000_CN_180757892_500000/RConn2 -- _CN_180757892_500000_CN_259425260_500000/RConn2
  _CN_253523129_500000_CN_180757892_500000/RConn3 -- T_180757892__Subestação_Samambaia/LConn3 -- _CN_154975532_500000_CN_180757892_500000/RConn3 -- _CN_283488616_500000_CN_180757892_500000/RConn3 -- _CN_180757892_500000_CN_259425260_500000/RConn3 -- bus319/LConn1
  _CN_32302779_500000_CN_32300871_500000/LConn1 -- T_32302779__/LConn1 -- _CN_32302779_500000_CN_32236291_500000/LConn1
  _CN_32302779_500000_CN_32300871_500000/LConn2 -- T_32302779__/LConn2 -- _CN_32302779_500000_CN_32236291_500000/LConn2
  _CN_32302779_500000_CN_32300871_500000/LConn3 -- T_32302779__/LConn3 -- _CN_32302779_500000_CN_32236291_500000/LConn3 -- bus320/LConn1
  _CN_32302779_500000_CN_32300871_500000/RConn1 -- T_32300871__Furnas/RConn1 -- _CN_32300871_500000_CN_32236291_500000/LConn1 -- L_32300871/LConn1
  _CN_32302779_500000_CN_32300871_500000/RConn2 -- T_32300871__Furnas/RConn2 -- _CN_32300871_500000_CN_32236291_500000/LConn2 -- L_32300871/LConn2
  _CN_32302779_500000_CN_32300871_500000/RConn3 -- T_32300871__Furnas/RConn3 -- _CN_32300871_500000_CN_32236291_500000/LConn3 -- L_32300871/LConn3 -- bus321/LConn1
  _CN_32302779_500000_CN_32236291_500000/RConn1 -- G_32236291_Usina_Hidrelétrica_de_Itaipu/RConn1 -- _CN_32300871_500000_CN_32236291_500000/RConn1
  _CN_32302779_500000_CN_32236291_500000/RConn2 -- G_32236291_Usina_Hidrelétrica_de_Itaipu/RConn2 -- _CN_32300871_500000_CN_32236291_500000/RConn2
  _CN_32302779_500000_CN_32236291_500000/RConn3 -- G_32236291_Usina_Hidrelétrica_de_Itaipu/RConn3 -- _CN_32300871_500000_CN_32236291_500000/RConn3 -- bus322/LConn1
  _CN_196020936_500000_CN_271242661_500000/LConn1 -- T_196020936__/LConn1 -- _CN_196020936_500000_CN_263232825_500000/RConn1
  _CN_196020936_500000_CN_271242661_500000/LConn2 -- T_196020936__/LConn2 -- _CN_196020936_500000_CN_263232825_500000/RConn2
  _CN_196020936_500000_CN_271242661_500000/LConn3 -- T_196020936__/LConn3 -- _CN_196020936_500000_CN_263232825_500000/RConn3 -- bus323/LConn1
  _CN_196020936_500000_CN_271242661_500000/RConn1 -- T_271242661__Subestação_Ribeiro_Gonçalves/LConn1 -- Colinas_Sobradinho_CN_271191830_500000_CN_271242661_500000/RConn1
  _CN_196020936_500000_CN_271242661_500000/RConn2 -- T_271242661__Subestação_Ribeiro_Gonçalves/LConn2 -- Colinas_Sobradinho_CN_271191830_500000_CN_271242661_500000/RConn2
  _CN_196020936_500000_CN_271242661_500000/RConn3 -- T_271242661__Subestação_Ribeiro_Gonçalves/LConn3 -- Colinas_Sobradinho_CN_271191830_500000_CN_271242661_500000/RConn3 -- bus324/LConn1
  T_216693990__/LConn1 -- Cachoeira_Paulista___Adrianópolis_CN_216693990_500000_CN_91627969_500000/LConn1
  T_216693990__/LConn2 -- Cachoeira_Paulista___Adrianópolis_CN_216693990_500000_CN_91627969_500000/LConn2
  Cachoeira_Paulista___Adrianópolis_CN_216693990_500000_CN_91627969_500000/LConn3 -- T_216693990__/LConn3 -- bus325/LConn1
  Cachoeira_Paulista___Adrianópolis_CN_216693990_500000_CN_91627969_500000/RConn1 -- T_91627969__Subestação_Adrianópolis/LConn1 -- UTE_Baixada_Fluminense___Seccionamento_Cachoeira_Paulista___Adrianópolis_CN_380022067_500000_CN_91627969_500000/LConn1 -- _CN_91627969_500000_CN_108224468_500000/LConn1
  Cachoeira_Paulista___Adrianópolis_CN_216693990_500000_CN_91627969_500000/RConn2 -- T_91627969__Subestação_Adrianópolis/LConn2 -- UTE_Baixada_Fluminense___Seccionamento_Cachoeira_Paulista___Adrianópolis_CN_380022067_500000_CN_91627969_500000/LConn2 -- _CN_91627969_500000_CN_108224468_500000/LConn2
  Cachoeira_Paulista___Adrianópolis_CN_216693990_500000_CN_91627969_500000/RConn3 -- T_91627969__Subestação_Adrianópolis/LConn3 -- UTE_Baixada_Fluminense___Seccionamento_Cachoeira_Paulista___Adrianópolis_CN_380022067_500000_CN_91627969_500000/LConn3 -- _CN_91627969_500000_CN_108224468_500000/LConn3 -- bus326/LConn1
  _CN_174906606_500000_CN_217292707_500000/LConn1 -- T_174906606__/LConn1 -- _CN_174906606_500000_CN_174852067_500000/LConn1
  _CN_174906606_500000_CN_217292707_500000/LConn2 -- T_174906606__/LConn2 -- _CN_174906606_500000_CN_174852067_500000/LConn2
  _CN_174906606_500000_CN_217292707_500000/LConn3 -- T_174906606__/LConn3 -- _CN_174906606_500000_CN_174852067_500000/LConn3 -- bus327/LConn1
  _CN_174906606_500000_CN_217292707_500000/RConn1 -- T_217292707__/LConn1 -- LT_São_Simão___Jaguara_CN_154030807_500000_CN_217292707_500000/RConn1
  _CN_174906606_500000_CN_217292707_500000/RConn2 -- T_217292707__/LConn2 -- LT_São_Simão___Jaguara_CN_154030807_500000_CN_217292707_500000/RConn2
  _CN_174906606_500000_CN_217292707_500000/RConn3 -- T_217292707__/LConn3 -- LT_São_Simão___Jaguara_CN_154030807_500000_CN_217292707_500000/RConn3 -- bus328/LConn1
  T_174852067__/LConn1 -- _CN_174906606_500000_CN_174852067_500000/RConn1
  T_174852067__/LConn2 -- _CN_174906606_500000_CN_174852067_500000/RConn2
  _CN_174906606_500000_CN_174852067_500000/RConn3 -- T_174852067__/LConn3 -- bus329/LConn1
  G_151624015_Governador_Bento_Munhoz_da_Rocha_Neto_(Foz_do_Areia)/RConn1 -- _CN_316971776_500000_CN_151624015_500000/RConn1
  G_151624015_Governador_Bento_Munhoz_da_Rocha_Neto_(Foz_do_Areia)/RConn2 -- _CN_316971776_500000_CN_151624015_500000/RConn2
  _CN_316971776_500000_CN_151624015_500000/RConn3 -- G_151624015_Governador_Bento_Munhoz_da_Rocha_Neto_(Foz_do_Areia)/RConn3 -- bus330/LConn1
  C3_CN_253692682_500000_CN_198634993_500000/RConn1 -- T_198634993__/LConn1 -- _CN_271191830_500000_CN_198634993_500000/RConn1 -- _CN_295701344_500000_CN_198634993_500000/LConn1
  C3_CN_253692682_500000_CN_198634993_500000/RConn2 -- T_198634993__/LConn2 -- _CN_271191830_500000_CN_198634993_500000/RConn2 -- _CN_295701344_500000_CN_198634993_500000/LConn2
  C3_CN_253692682_500000_CN_198634993_500000/RConn3 -- T_198634993__/LConn3 -- _CN_271191830_500000_CN_198634993_500000/RConn3 -- _CN_295701344_500000_CN_198634993_500000/LConn3 -- bus331/LConn1
  T_302931307_440000_LT_Água_Vermelha/LConn1 -- _CN_154030807_500000_CN_302931307_500000/RConn1
  T_302931307_440000_LT_Água_Vermelha/LConn2 -- _CN_154030807_500000_CN_302931307_500000/RConn2
  _CN_154030807_500000_CN_302931307_500000/RConn3 -- T_302931307_440000_LT_Água_Vermelha/LConn3 -- bus332/LConn1
  _CN_154030807_500000_CN_390650772_500000/RConn1 -- G_390650772_UHE_Itumbiara/RConn1 -- _CN_154975532_500000_CN_390650772_500000/RConn1
  _CN_154030807_500000_CN_390650772_500000/RConn2 -- G_390650772_UHE_Itumbiara/RConn2 -- _CN_154975532_500000_CN_390650772_500000/RConn2
  _CN_154030807_500000_CN_390650772_500000/RConn3 -- G_390650772_UHE_Itumbiara/RConn3 -- _CN_154975532_500000_CN_390650772_500000/RConn3 -- bus333/LConn1
  _CN_280057613_500000_CN_390650773_500000/LConn1 -- T_280057613__Subestação_de_Xingó___CHESF/LConn1 -- _CN_280057613_500000_CN_247537019_500000/LConn1
  _CN_280057613_500000_CN_390650773_500000/LConn2 -- T_280057613__Subestação_de_Xingó___CHESF/LConn2 -- _CN_280057613_500000_CN_247537019_500000/LConn2
  _CN_280057613_500000_CN_390650773_500000/LConn3 -- T_280057613__Subestação_de_Xingó___CHESF/LConn3 -- _CN_280057613_500000_CN_247537019_500000/LConn3 -- bus334/LConn1
  G_390650773_UHE_Xingó/RConn1 -- _CN_280057613_500000_CN_390650773_500000/RConn1
  G_390650773_UHE_Xingó/RConn2 -- _CN_280057613_500000_CN_390650773_500000/RConn2
  _CN_280057613_500000_CN_390650773_500000/RConn3 -- G_390650773_UHE_Xingó/RConn3 -- bus335/LConn1
  _CN_280057613_500000_CN_247537019_500000/RConn1 -- T_247537019__Subestação_CROP/LConn1 -- _CN_247537019_500000_CN_390650768_500000/RConn1
  _CN_280057613_500000_CN_247537019_500000/RConn2 -- T_247537019__Subestação_CROP/LConn2 -- _CN_247537019_500000_CN_390650768_500000/RConn2
  _CN_280057613_500000_CN_247537019_500000/RConn3 -- T_247537019__Subestação_CROP/LConn3 -- _CN_247537019_500000_CN_390650768_500000/RConn3 -- bus336/LConn1
  T_304658726__/LConn1 -- _CN_304658726_500000_CN_271524307_500000/RConn1
  T_304658726__/LConn2 -- _CN_304658726_500000_CN_271524307_500000/RConn2
  _CN_304658726_500000_CN_271524307_500000/RConn3 -- T_304658726__/LConn3 -- bus337/LConn1
  T_129484075__Subestação_de_Furnas/LConn1 -- _CN_129484075_500000_CN_171525050_500000/RConn1
  T_129484075__Subestação_de_Furnas/LConn2 -- _CN_129484075_500000_CN_171525050_500000/RConn2
  _CN_129484075_500000_CN_171525050_500000/RConn3 -- T_129484075__Subestação_de_Furnas/LConn3 -- bus338/LConn1
  T_380022067__/LConn1 -- UTE_Baixada_Fluminense___Seccionamento_Cachoeira_Paulista___Adrianópolis_CN_380022067_500000_CN_91627969_500000/RConn1
  T_380022067__/LConn2 -- UTE_Baixada_Fluminense___Seccionamento_Cachoeira_Paulista___Adrianópolis_CN_380022067_500000_CN_91627969_500000/RConn2
  UTE_Baixada_Fluminense___Seccionamento_Cachoeira_Paulista___Adrianópolis_CN_380022067_500000_CN_91627969_500000/RConn3 -- T_380022067__/LConn3 -- bus339/LConn1
  G_304144597_/RConn1 -- _CN_304139576_500000_CN_304144597_500000/RConn1
  G_304144597_/RConn2 -- _CN_304139576_500000_CN_304144597_500000/RConn2
  _CN_304139576_500000_CN_304144597_500000/RConn3 -- G_304144597_/RConn3 -- bus340/LConn1
  _CN_283510602_500000_CN_297523069_500000/RConn1 -- T_283510602__Subestação_de_São_Gotardo/LConn1 -- Emborcação___São_Gotardo_CN_283510602_500000_CN_283488616_500000/RConn1
  _CN_283510602_500000_CN_297523069_500000/RConn2 -- T_283510602__Subestação_de_São_Gotardo/LConn2 -- Emborcação___São_Gotardo_CN_283510602_500000_CN_283488616_500000/RConn2
  _CN_283510602_500000_CN_297523069_500000/RConn3 -- T_283510602__Subestação_de_São_Gotardo/LConn3 -- Emborcação___São_Gotardo_CN_283510602_500000_CN_283488616_500000/RConn3 -- bus341/LConn1
  T_293811021__Subestação_Ibicoara/LConn1 -- Linha_de_Transmissão_Norte___Nordeste_CN_293811021_500000_CN_293729126_500000/RConn1
  T_293811021__Subestação_Ibicoara/LConn2 -- Linha_de_Transmissão_Norte___Nordeste_CN_293811021_500000_CN_293729126_500000/RConn2
  Linha_de_Transmissão_Norte___Nordeste_CN_293811021_500000_CN_293729126_500000/RConn3 -- T_293811021__Subestação_Ibicoara/LConn3 -- bus342/LConn1
  T_295701344__/LConn1 -- _CN_295701344_500000_CN_198634993_500000/RConn1
  T_295701344__/LConn2 -- _CN_295701344_500000_CN_198634993_500000/RConn2
  _CN_295701344_500000_CN_198634993_500000/RConn3 -- T_295701344__/LConn3 -- bus343/LConn1
  G_295766704_UHE_Emborcação/RConn1 -- _CN_283488616_500000_CN_295766704_500000/RConn1
  G_295766704_UHE_Emborcação/RConn2 -- _CN_283488616_500000_CN_295766704_500000/RConn2
  _CN_283488616_500000_CN_295766704_500000/RConn3 -- G_295766704_UHE_Emborcação/RConn3 -- bus344/LConn1
  _CN_125761911_500000_CN_125761912_500000/RConn1 -- T_125761912_750000_/RConn1 -- L_125761912/LConn1
  _CN_125761911_500000_CN_125761912_500000/RConn2 -- T_125761912_750000_/RConn2 -- L_125761912/LConn2
  _CN_125761911_500000_CN_125761912_500000/RConn3 -- T_125761912_750000_/RConn3 -- L_125761912/LConn3 -- bus345/LConn1
  T_108224468_500000_Subestação_Grajaú/LConn1 -- _CN_91627969_500000_CN_108224468_500000/RConn1
  T_108224468_500000_Subestação_Grajaú/LConn2 -- _CN_91627969_500000_CN_108224468_500000/RConn2
  _CN_91627969_500000_CN_108224468_500000/RConn3 -- T_108224468_500000_Subestação_Grajaú/LConn3 -- bus346/LConn1
  T_215284729__/LConn1 -- _CN_215284729_500000_CN_215429821_500000/LConn1
  T_215284729__/LConn2 -- _CN_215284729_500000_CN_215429821_500000/LConn2
  _CN_215284729_500000_CN_215429821_500000/LConn3 -- T_215284729__/LConn3 -- bus347/LConn1
  G_215429821_UHE_de_Tucuruí/RConn1 -- _CN_215284729_500000_CN_215429821_500000/RConn1
  G_215429821_UHE_de_Tucuruí/RConn2 -- _CN_215284729_500000_CN_215429821_500000/RConn2
  _CN_215284729_500000_CN_215429821_500000/RConn3 -- G_215429821_UHE_de_Tucuruí/RConn3 -- bus348/LConn1
  _CN_125761912_750000_CN_202622375_750000/LConn1 -- T_125761912_750000_/LConn1 -- _CN_125761912_750000_CN_32300871_750000/LConn1
  _CN_125761912_750000_CN_202622375_750000/LConn2 -- T_125761912_750000_/LConn2 -- _CN_125761912_750000_CN_32300871_750000/LConn2
  _CN_125761912_750000_CN_202622375_750000/LConn3 -- T_125761912_750000_/LConn3 -- _CN_125761912_750000_CN_32300871_750000/LConn3 -- bus349/LConn1
  _CN_125761912_750000_CN_202622375_750000/RConn1 -- T_202622375__/LConn1 -- _CN_202622375_750000_CN_175909709_750000/LConn1
  _CN_125761912_750000_CN_202622375_750000/RConn2 -- T_202622375__/LConn2 -- _CN_202622375_750000_CN_175909709_750000/LConn2
  _CN_125761912_750000_CN_202622375_750000/RConn3 -- T_202622375__/LConn3 -- _CN_202622375_750000_CN_175909709_750000/LConn3 -- bus350/LConn1
  T_32300871__Furnas/LConn1 -- _CN_125761912_750000_CN_32300871_750000/RConn1
  T_32300871__Furnas/LConn2 -- _CN_125761912_750000_CN_32300871_750000/RConn2
  _CN_125761912_750000_CN_32300871_750000/RConn3 -- T_32300871__Furnas/LConn3 -- bus351/LConn1
  T_175909709__/LConn1 -- _CN_202622375_750000_CN_175909709_750000/RConn1
  T_175909709__/LConn2 -- _CN_202622375_750000_CN_175909709_750000/RConn2
  _CN_202622375_750000_CN_175909709_750000/RConn3 -- T_175909709__/LConn3 -- bus352/LConn1
  T_204662228__/RConn1 -- L_204662228/LConn1
  T_204662228__/RConn2 -- L_204662228/LConn2
  L_204662228/LConn3 -- T_204662228__/RConn3 -- bus353/LConn1
  T_208450687__Subestação_COPEL_Toledo/RConn1 -- L_208450687/LConn1
  T_208450687__Subestação_COPEL_Toledo/RConn2 -- L_208450687/LConn2
  L_208450687/LConn3 -- T_208450687__Subestação_COPEL_Toledo/RConn3 -- bus354/LConn1
  T_207573521__/RConn1 -- L_207573521/LConn1
  T_207573521__/RConn2 -- L_207573521/LConn2
  L_207573521/LConn3 -- T_207573521__/RConn3 -- bus355/LConn1
  T_430397465__Subestação_Rio_Azul/RConn1 -- L_430397465/LConn1
  T_430397465__Subestação_Rio_Azul/RConn2 -- L_430397465/LConn2
  L_430397465/LConn3 -- T_430397465__Subestação_Rio_Azul/RConn3 -- bus356/LConn1
  T_430390206__Subestação_Irati/RConn1 -- L_430390206/LConn1
  T_430390206__Subestação_Irati/RConn2 -- L_430390206/LConn2
  L_430390206/LConn3 -- T_430390206__Subestação_Irati/RConn3 -- bus357/LConn1
  T_171490852__Subestação_Parque_das_Emas/RConn1 -- L_171490852/LConn1
  T_171490852__Subestação_Parque_das_Emas/RConn2 -- L_171490852/LConn2
  L_171490852/LConn3 -- T_171490852__Subestação_Parque_das_Emas/RConn3 -- bus358/LConn1
  T_238221864__Subestação_Chapecó_II/RConn1 -- L_238221864/LConn1
  T_238221864__Subestação_Chapecó_II/RConn2 -- L_238221864/LConn2
  L_238221864/LConn3 -- T_238221864__Subestação_Chapecó_II/RConn3 -- bus359/LConn1
  T_206686475_138000_Subestação_Xanxerê_Celesc/RConn1 -- L_206686475/LConn1
  T_206686475_138000_Subestação_Xanxerê_Celesc/RConn2 -- L_206686475/LConn2
  L_206686475/LConn3 -- T_206686475_138000_Subestação_Xanxerê_Celesc/RConn3 -- bus360/LConn1
  T_206721069__Subestação_BRF/RConn1 -- L_206721069/LConn1
  T_206721069__Subestação_BRF/RConn2 -- L_206721069/LConn2
  L_206721069/LConn3 -- T_206721069__Subestação_BRF/RConn3 -- bus361/LConn1
  T_361161020__/RConn1 -- L_361161020/LConn1
  T_361161020__/RConn2 -- L_361161020/LConn2
  L_361161020/LConn3 -- T_361161020__/RConn3 -- bus362/LConn1
  T_166830130__/RConn1 -- L_166830130/LConn1
  T_166830130__/RConn2 -- L_166830130/LConn2
  L_166830130/LConn3 -- T_166830130__/RConn3 -- bus363/LConn1
  T_108479345__/RConn1 -- L_108479345/LConn1
  T_108479345__/RConn2 -- L_108479345/LConn2
  L_108479345/LConn3 -- T_108479345__/RConn3 -- bus364/LConn1
  T_283714330__/RConn1 -- L_283714330/LConn1
  T_283714330__/RConn2 -- L_283714330/LConn2
  L_283714330/LConn3 -- T_283714330__/RConn3 -- bus365/LConn1
  T_109816378__/RConn1 -- L_109816378/LConn1
  T_109816378__/RConn2 -- L_109816378/LConn2
  L_109816378/LConn3 -- T_109816378__/RConn3 -- bus366/LConn1
  T_179031106__/RConn1 -- L_179031106/LConn1
  T_179031106__/RConn2 -- L_179031106/LConn2
  L_179031106/LConn3 -- T_179031106__/RConn3 -- bus367/LConn1
  T_180585890_138000_/RConn1 -- L_180585890/LConn1
  T_180585890_138000_/RConn2 -- L_180585890/LConn2
  L_180585890/LConn3 -- T_180585890_138000_/RConn3 -- bus368/LConn1
  T_258563660__/RConn1 -- L_258563660/LConn1
  T_258563660__/RConn2 -- L_258563660/LConn2
  L_258563660/LConn3 -- T_258563660__/RConn3 -- bus369/LConn1
  T_374370399__/RConn1 -- L_374370399/LConn1
  T_374370399__/RConn2 -- L_374370399/LConn2
  L_374370399/LConn3 -- T_374370399__/RConn3 -- bus370/LConn1
  T_215501231__/RConn1 -- L_215501231/LConn1
  T_215501231__/RConn2 -- L_215501231/LConn2
  L_215501231/LConn3 -- T_215501231__/RConn3 -- bus371/LConn1
  T_169845345__Subestação_Rodoviária/RConn1 -- L_169845345/LConn1
  T_169845345__Subestação_Rodoviária/RConn2 -- L_169845345/LConn2
  L_169845345/LConn3 -- T_169845345__Subestação_Rodoviária/RConn3 -- bus372/LConn1
  T_167892676__Subestação_CPA/RConn1 -- L_167892676/LConn1
  T_167892676__Subestação_CPA/RConn2 -- L_167892676/LConn2
  L_167892676/LConn3 -- T_167892676__Subestação_CPA/RConn3 -- bus373/LConn1
  T_315151458__Daia/RConn1 -- L_315151458/LConn1
  T_315151458__Daia/RConn2 -- L_315151458/LConn2
  L_315151458/LConn3 -- T_315151458__Daia/RConn3 -- bus374/LConn1
  T_315172147__/RConn1 -- L_315172147/LConn1
  T_315172147__/RConn2 -- L_315172147/LConn2
  L_315172147/LConn3 -- T_315172147__/RConn3 -- bus375/LConn1
  T_168904821__Jauru/RConn1 -- L_168904821/LConn1
  T_168904821__Jauru/RConn2 -- L_168904821/LConn2
  L_168904821/LConn3 -- T_168904821__Jauru/RConn3 -- bus376/LConn1
  T_306676350__Subestação_Batávia/RConn1 -- L_306676350/LConn1
  T_306676350__Subestação_Batávia/RConn2 -- L_306676350/LConn2
  L_306676350/LConn3 -- T_306676350__Subestação_Batávia/RConn3 -- bus377/LConn1
  T_168904839__Subestação_Guaporé/RConn1 -- L_168904839/LConn1
  T_168904839__Subestação_Guaporé/RConn2 -- L_168904839/LConn2
  L_168904839/LConn3 -- T_168904839__Subestação_Guaporé/RConn3 -- bus378/LConn1
  T_168933874__/RConn1 -- L_168933874/LConn1
  T_168933874__/RConn2 -- L_168933874/LConn2
  L_168933874/LConn3 -- T_168933874__/RConn3 -- bus379/LConn1
  T_290054123__São_Luís/RConn1 -- L_290054123/LConn1
  T_290054123__São_Luís/RConn2 -- L_290054123/LConn2
  L_290054123/LConn3 -- T_290054123__São_Luís/RConn3 -- bus380/LConn1
  T_288144022__/RConn1 -- L_288144022/LConn1
  T_288144022__/RConn2 -- L_288144022/LConn2
  L_288144022/LConn3 -- T_288144022__/RConn3 -- bus381/LConn1
  T_315069128__Jundiai/RConn1 -- L_315069128/LConn1
  T_315069128__Jundiai/RConn2 -- L_315069128/LConn2
  L_315069128/LConn3 -- T_315069128__Jundiai/RConn3 -- bus382/LConn1
  T_286116282__/RConn1 -- L_286116282/LConn1
  T_286116282__/RConn2 -- L_286116282/LConn2
  L_286116282/LConn3 -- T_286116282__/RConn3 -- bus383/LConn1
  T_313920196__/RConn1 -- L_313920196/LConn1
  T_313920196__/RConn2 -- L_313920196/LConn2
  L_313920196/LConn3 -- T_313920196__/RConn3 -- bus384/LConn1
  T_108435010__/RConn1 -- L_108435010/LConn1
  T_108435010__/RConn2 -- L_108435010/LConn2
  L_108435010/LConn3 -- T_108435010__/RConn3 -- bus385/LConn1
  T_179642046__Subestação_Mourão/RConn1 -- L_179642046/LConn1
  T_179642046__Subestação_Mourão/RConn2 -- L_179642046/LConn2
  L_179642046/LConn3 -- T_179642046__Subestação_Mourão/RConn3 -- bus386/LConn1
  T_167284528__Subestação_EPE/RConn1 -- L_167284528/LConn1
  T_167284528__Subestação_EPE/RConn2 -- L_167284528/LConn2
  L_167284528/LConn3 -- T_167284528__Subestação_EPE/RConn3 -- bus387/LConn1
  T_171490850__Subestação_Couto_Magalhães/RConn1 -- L_171490850/LConn1
  T_171490850__Subestação_Couto_Magalhães/RConn2 -- L_171490850/LConn2
  L_171490850/LConn3 -- T_171490850__Subestação_Couto_Magalhães/RConn3 -- bus388/LConn1
  T_199921358__/RConn1 -- L_199921358/LConn1
  T_199921358__/RConn2 -- L_199921358/LConn2
  L_199921358/LConn3 -- T_199921358__/RConn3 -- bus389/LConn1
  T_199921360__/RConn1 -- L_199921360/LConn1
  T_199921360__/RConn2 -- L_199921360/LConn2
  L_199921360/LConn3 -- T_199921360__/RConn3 -- bus390/LConn1
  T_200365032__/RConn1 -- L_200365032/LConn1
  T_200365032__/RConn2 -- L_200365032/LConn2
  L_200365032/LConn3 -- T_200365032__/RConn3 -- bus391/LConn1
  T_194362821__Santa_Maria_1/RConn1 -- L_194362821/LConn1
  T_194362821__Santa_Maria_1/RConn2 -- L_194362821/LConn2
  L_194362821/LConn3 -- T_194362821__Santa_Maria_1/RConn3 -- bus392/LConn1
  T_178582739__Subestação_Canarana/RConn1 -- L_178582739/LConn1
  T_178582739__Subestação_Canarana/RConn2 -- L_178582739/LConn2
  L_178582739/LConn3 -- T_178582739__Subestação_Canarana/RConn3 -- bus393/LConn1
  T_178582740__Subestação_Querência/RConn1 -- L_178582740/LConn1
  T_178582740__Subestação_Querência/RConn2 -- L_178582740/LConn2
  L_178582740/LConn3 -- T_178582740__Subestação_Querência/RConn3 -- bus394/LConn1
  T_154646743__/RConn1 -- L_154646743/LConn1
  T_154646743__/RConn2 -- L_154646743/LConn2
  L_154646743/LConn3 -- T_154646743__/RConn3 -- bus395/LConn1
  T_256782585__/RConn1 -- L_256782585/LConn1
  T_256782585__/RConn2 -- L_256782585/LConn2
  L_256782585/LConn3 -- T_256782585__/RConn3 -- bus396/LConn1
  T_176682224__Subestação_Cristo_Rei/RConn1 -- L_176682224/LConn1
  T_176682224__Subestação_Cristo_Rei/RConn2 -- L_176682224/LConn2
  L_176682224/LConn3 -- T_176682224__Subestação_Cristo_Rei/RConn3 -- bus397/LConn1
  T_32957294__/RConn1 -- L_32957294/LConn1
  T_32957294__/RConn2 -- L_32957294/LConn2
  L_32957294/LConn3 -- T_32957294__/RConn3 -- bus398/LConn1
  T_112451827__/RConn1 -- L_112451827/LConn1
  T_112451827__/RConn2 -- L_112451827/LConn2
  L_112451827/LConn3 -- T_112451827__/RConn3 -- bus399/LConn1
  T_111514032__/RConn1 -- L_111514032/LConn1
  T_111514032__/RConn2 -- L_111514032/LConn2
  L_111514032/LConn3 -- T_111514032__/RConn3 -- bus400/LConn1
  T_430385951__Subestação_Guarapuava/RConn1 -- L_430385951/LConn1
  T_430385951__Subestação_Guarapuava/RConn2 -- L_430385951/LConn2
  L_430385951/LConn3 -- T_430385951__Subestação_Guarapuava/RConn3 -- bus401/LConn1
  T_177544973__Subestação_de_Paranatinga/RConn1 -- L_177544973/LConn1
  T_177544973__Subestação_de_Paranatinga/RConn2 -- L_177544973/LConn2
  L_177544973/LConn3 -- T_177544973__Subestação_de_Paranatinga/RConn3 -- bus402/LConn1
  T_177544975__Subestação_Primavera_do_Leste/RConn1 -- L_177544975/LConn1
  T_177544975__Subestação_Primavera_do_Leste/RConn2 -- L_177544975/LConn2
  L_177544975/LConn3 -- T_177544975__Subestação_Primavera_do_Leste/RConn3 -- bus403/LConn1
  T_396009895_138000_Subestação_Jardim_Tropical/RConn1 -- L_396009895/LConn1
  T_396009895_138000_Subestação_Jardim_Tropical/RConn2 -- L_396009895/LConn2
  L_396009895/LConn3 -- T_396009895_138000_Subestação_Jardim_Tropical/RConn3 -- bus404/LConn1
  T_129482585_138000_Subestação_Jardim_Alvorada/RConn1 -- L_129482585/LConn1
  T_129482585_138000_Subestação_Jardim_Alvorada/RConn2 -- L_129482585/LConn2
  L_129482585/LConn3 -- T_129482585_138000_Subestação_Jardim_Alvorada/RConn3 -- bus405/LConn1
  T_173329706__/RConn1 -- L_173329706/LConn1
  T_173329706__/RConn2 -- L_173329706/LConn2
  L_173329706/LConn3 -- T_173329706__/RConn3 -- bus406/LConn1
  T_430403964__Subestação_Sabará/RConn1 -- L_430403964/LConn1
  T_430403964__Subestação_Sabará/RConn2 -- L_430403964/LConn2
  L_430403964/LConn3 -- T_430403964__Subestação_Sabará/RConn3 -- bus407/LConn1
  T_395653952__Subestação_Barbosa_Ferraz/RConn1 -- L_395653952/LConn1
  T_395653952__Subestação_Barbosa_Ferraz/RConn2 -- L_395653952/LConn2
  L_395653952/LConn3 -- T_395653952__Subestação_Barbosa_Ferraz/RConn3 -- bus408/LConn1
  T_395653957__Subestação_Mamborê/RConn1 -- L_395653957/LConn1
  T_395653957__Subestação_Mamborê/RConn2 -- L_395653957/LConn2
  L_395653957/LConn3 -- T_395653957__Subestação_Mamborê/RConn3 -- bus409/LConn1
  T_395793739_138000_Subestação_Mandacaru/RConn1 -- L_395793739/LConn1
  T_395793739_138000_Subestação_Mandacaru/RConn2 -- L_395793739/LConn2
  L_395793739/LConn3 -- T_395793739_138000_Subestação_Mandacaru/RConn3 -- bus410/LConn1
  T_405782885__Subestação_de_Pombal/RConn1 -- L_405782885/LConn1
  T_405782885__Subestação_de_Pombal/RConn2 -- L_405782885/LConn2
  L_405782885/LConn3 -- T_405782885__Subestação_de_Pombal/RConn3 -- bus411/LConn1
  T_398070144__Subestação_de_Jericó/RConn1 -- L_398070144/LConn1
  T_398070144__Subestação_de_Jericó/RConn2 -- L_398070144/LConn2
  L_398070144/LConn3 -- T_398070144__Subestação_de_Jericó/RConn3 -- bus412/LConn1
  T_280699285__/RConn1 -- L_280699285/LConn1
  T_280699285__/RConn2 -- L_280699285/LConn2
  L_280699285/LConn3 -- T_280699285__/RConn3 -- bus413/LConn1
  T_280699287__/RConn1 -- L_280699287/LConn1
  T_280699287__/RConn2 -- L_280699287/LConn2
  L_280699287/LConn3 -- T_280699287__/RConn3 -- bus414/LConn1
  T_122252210__/RConn1 -- L_122252210/LConn1
  T_122252210__/RConn2 -- L_122252210/LConn2
  L_122252210/LConn3 -- T_122252210__/RConn3 -- bus415/LConn1
  T_122252211__/RConn1 -- L_122252211/LConn1
  T_122252211__/RConn2 -- L_122252211/LConn2
  L_122252211/LConn3 -- T_122252211__/RConn3 -- bus416/LConn1
  T_168692185__/RConn1 -- L_168692185/LConn1
  T_168692185__/RConn2 -- L_168692185/LConn2
  L_168692185/LConn3 -- T_168692185__/RConn3 -- bus417/LConn1
  T_108435903__Substação_Frei_Caneca/RConn1 -- L_108435903/LConn1
  T_108435903__Substação_Frei_Caneca/RConn2 -- L_108435903/LConn2
  L_108435903/LConn3 -- T_108435903__Substação_Frei_Caneca/RConn3 -- bus418/LConn1
  T_312985603__Subestação_Nova_Mutum/RConn1 -- L_312985603/LConn1
  T_312985603__Subestação_Nova_Mutum/RConn2 -- L_312985603/LConn2
  L_312985603/LConn3 -- T_312985603__Subestação_Nova_Mutum/RConn3 -- bus419/LConn1
  T_171732983__Subestação_Sorriso/RConn1 -- L_171732983/LConn1
  T_171732983__Subestação_Sorriso/RConn2 -- L_171732983/LConn2
  L_171732983/LConn3 -- T_171732983__Subestação_Sorriso/RConn3 -- bus420/LConn1
  T_171732980__Subestação_Lucas_do_Rio_Verde/RConn1 -- L_171732980/LConn1
  T_171732980__Subestação_Lucas_do_Rio_Verde/RConn2 -- L_171732980/LConn2
  L_171732980/LConn3 -- T_171732980__Subestação_Lucas_do_Rio_Verde/RConn3 -- bus421/LConn1
  T_240522248__CHESF/RConn1 -- L_240522248/LConn1
  T_240522248__CHESF/RConn2 -- L_240522248/LConn2
  L_240522248/LConn3 -- T_240522248__CHESF/RConn3 -- bus422/LConn1
  T_262122922__Subestação_de_Russas/RConn1 -- L_262122922/LConn1
  T_262122922__Subestação_de_Russas/RConn2 -- L_262122922/LConn2
  L_262122922/LConn3 -- T_262122922__Subestação_de_Russas/RConn3 -- bus423/LConn1
  T_261953891__/RConn1 -- L_261953891/LConn1
  T_261953891__/RConn2 -- L_261953891/LConn2
  L_261953891/LConn3 -- T_261953891__/RConn3 -- bus424/LConn1
  T_204336141__/RConn1 -- L_204336141/LConn1
  T_204336141__/RConn2 -- L_204336141/LConn2
  L_204336141/LConn3 -- T_204336141__/RConn3 -- bus425/LConn1
  T_194446718__Santa_Maria_3/RConn1 -- L_194446718/LConn1
  T_194446718__Santa_Maria_3/RConn2 -- L_194446718/LConn2
  L_194446718/LConn3 -- T_194446718__Santa_Maria_3/RConn3 -- bus426/LConn1
  T_146723856_230000_Subestação_Maringá/RConn1 -- L_146723856/LConn1
  T_146723856_230000_Subestação_Maringá/RConn2 -- L_146723856/LConn2
  L_146723856/LConn3 -- T_146723856_230000_Subestação_Maringá/RConn3 -- bus427/LConn1
  T_303915320__/RConn1 -- L_303915320/LConn1
  T_303915320__/RConn2 -- L_303915320/LConn2
  L_303915320/LConn3 -- T_303915320__/RConn3 -- bus428/LConn1
  T_262826015__/RConn1 -- L_262826015/LConn1
  T_262826015__/RConn2 -- L_262826015/LConn2
  L_262826015/LConn3 -- T_262826015__/RConn3 -- bus429/LConn1
  T_241914909__/RConn1 -- L_241914909/LConn1
  T_241914909__/RConn2 -- L_241914909/LConn2
  L_241914909/LConn3 -- T_241914909__/RConn3 -- bus430/LConn1
  T_242506209__/RConn1 -- L_242506209/LConn1
  T_242506209__/RConn2 -- L_242506209/LConn2
  L_242506209/LConn3 -- T_242506209__/RConn3 -- bus431/LConn1
  T_241914935__/RConn1 -- L_241914935/LConn1
  T_241914935__/RConn2 -- L_241914935/LConn2
  L_241914935/LConn3 -- T_241914935__/RConn3 -- bus432/LConn1
  T_242506367__/RConn1 -- L_242506367/LConn1
  T_242506367__/RConn2 -- L_242506367/LConn2
  L_242506367/LConn3 -- T_242506367__/RConn3 -- bus433/LConn1
  T_171490854__Subestação_UHE_Itiquira/RConn1 -- L_171490854/LConn1
  T_171490854__Subestação_UHE_Itiquira/RConn2 -- L_171490854/LConn2
  L_171490854/LConn3 -- T_171490854__Subestação_UHE_Itiquira/RConn3 -- bus434/LConn1
  T_291608487__/RConn1 -- L_291608487/LConn1
  T_291608487__/RConn2 -- L_291608487/LConn2
  L_291608487/LConn3 -- T_291608487__/RConn3 -- bus435/LConn1
  T_282046525__Subestação_de_energia_elétrica_de_Itaituba/RConn1 -- L_282046525/LConn1
  T_282046525__Subestação_de_energia_elétrica_de_Itaituba/RConn2 -- L_282046525/LConn2
  L_282046525/LConn3 -- T_282046525__Subestação_de_energia_elétrica_de_Itaituba/RConn3 -- bus436/LConn1
  T_320566584__/RConn1 -- L_320566584/LConn1
  T_320566584__/RConn2 -- L_320566584/LConn2
  L_320566584/LConn3 -- T_320566584__/RConn3 -- bus437/LConn1
  T_306908735__Subestação_Barreiras/RConn1 -- L_306908735/LConn1
  T_306908735__Subestação_Barreiras/RConn2 -- L_306908735/LConn2
  L_306908735/LConn3 -- T_306908735__Subestação_Barreiras/RConn3 -- bus438/LConn1
  T_320600566__/RConn1 -- L_320600566/LConn1
  T_320600566__/RConn2 -- L_320600566/LConn2
  L_320600566/LConn3 -- T_320600566__/RConn3 -- bus439/LConn1
  T_105361984__/RConn1 -- L_105361984/LConn1
  T_105361984__/RConn2 -- L_105361984/LConn2
  L_105361984/LConn3 -- T_105361984__/RConn3 -- bus440/LConn1
  T_199918657__/RConn1 -- L_199918657/LConn1
  T_199918657__/RConn2 -- L_199918657/LConn2
  L_199918657/LConn3 -- T_199918657__/RConn3 -- bus441/LConn1
  T_200489312__Passo_Real/RConn1 -- L_200489312/LConn1
  T_200489312__Passo_Real/RConn2 -- L_200489312/LConn2
  L_200489312/LConn3 -- T_200489312__Passo_Real/RConn3 -- bus442/LConn1
  T_271789127__Subestação_De_Porto_Velho/RConn1 -- L_271789127/LConn1
  T_271789127__Subestação_De_Porto_Velho/RConn2 -- L_271789127/LConn2
  L_271789127/LConn3 -- T_271789127__Subestação_De_Porto_Velho/RConn3 -- bus443/LConn1
  T_232080998__/RConn1 -- L_232080998/LConn1
  T_232080998__/RConn2 -- L_232080998/LConn2
  L_232080998/LConn3 -- T_232080998__/RConn3 -- bus444/LConn1
  T_253518922__/RConn1 -- L_253518922/LConn1
  T_253518922__/RConn2 -- L_253518922/LConn2
  L_253518922/LConn3 -- T_253518922__/RConn3 -- bus445/LConn1
  T_253296634__/RConn1 -- L_253296634/LConn1
  T_253296634__/RConn2 -- L_253296634/LConn2
  L_253296634/LConn3 -- T_253296634__/RConn3 -- bus446/LConn1
  T_251440816__/RConn1 -- L_251440816/LConn1
  T_251440816__/RConn2 -- L_251440816/LConn2
  L_251440816/LConn3 -- T_251440816__/RConn3 -- bus447/LConn1
  T_171063374__/RConn1 -- L_171063374/LConn1
  T_171063374__/RConn2 -- L_171063374/LConn2
  L_171063374/LConn3 -- T_171063374__/RConn3 -- bus448/LConn1
  T_200004360__Substação_Palhoça/RConn1 -- L_200004360/LConn1
  T_200004360__Substação_Palhoça/RConn2 -- L_200004360/LConn2
  L_200004360/LConn3 -- T_200004360__Substação_Palhoça/RConn3 -- bus449/LConn1
  T_260344421__Subestação_Brasnorte/RConn1 -- L_260344421/LConn1
  T_260344421__Subestação_Brasnorte/RConn2 -- L_260344421/LConn2
  L_260344421/LConn3 -- T_260344421__Subestação_Brasnorte/RConn3 -- bus450/LConn1
  T_313073391__/RConn1 -- L_313073391/LConn1
  T_313073391__/RConn2 -- L_313073391/LConn2
  L_313073391/LConn3 -- T_313073391__/RConn3 -- bus451/LConn1
  T_260845415__Subestação_Barra_do_Peixe/RConn1 -- L_260845415/LConn1
  T_260845415__Subestação_Barra_do_Peixe/RConn2 -- L_260845415/LConn2
  L_260845415/LConn3 -- T_260845415__Subestação_Barra_do_Peixe/RConn3 -- bus452/LConn1
  T_253509480__/RConn1 -- L_253509480/LConn1
  T_253509480__/RConn2 -- L_253509480/LConn2
  L_253509480/LConn3 -- T_253509480__/RConn3 -- bus453/LConn1
  T_237588091_230000_/RConn1 -- L_237588091/LConn1
  T_237588091_230000_/RConn2 -- L_237588091/LConn2
  L_237588091/LConn3 -- T_237588091_230000_/RConn3 -- bus454/LConn1
  T_172447363__/RConn1 -- L_172447363/LConn1
  T_172447363__/RConn2 -- L_172447363/LConn2
  L_172447363/LConn3 -- T_172447363__/RConn3 -- bus455/LConn1
  T_320709254__/RConn1 -- L_320709254/LConn1
  T_320709254__/RConn2 -- L_320709254/LConn2
  L_320709254/LConn3 -- T_320709254__/RConn3 -- bus456/LConn1
  T_255983102__/RConn1 -- L_255983102/LConn1
  T_255983102__/RConn2 -- L_255983102/LConn2
  L_255983102/LConn3 -- T_255983102__/RConn3 -- bus457/LConn1
  T_253338257__/RConn1 -- L_253338257/LConn1
  T_253338257__/RConn2 -- L_253338257/LConn2
  L_253338257/LConn3 -- T_253338257__/RConn3 -- bus458/LConn1
  T_276741266__/RConn1 -- L_276741266/LConn1
  T_276741266__/RConn2 -- L_276741266/LConn2
  L_276741266/LConn3 -- T_276741266__/RConn3 -- bus459/LConn1
  T_161482453_230000_Subestação_Manaus/RConn1 -- L_161482453/LConn1
  T_161482453_230000_Subestação_Manaus/RConn2 -- L_161482453/LConn2
  L_161482453/LConn3 -- T_161482453_230000_Subestação_Manaus/RConn3 -- bus460/LConn1
  T_131689631__/RConn1 -- L_131689631/LConn1
  T_131689631__/RConn2 -- L_131689631/LConn2
  L_131689631/LConn3 -- T_131689631__/RConn3 -- bus461/LConn1
  T_150728362__/RConn1 -- L_150728362/LConn1
  T_150728362__/RConn2 -- L_150728362/LConn2
  L_150728362/LConn3 -- T_150728362__/RConn3 -- bus462/LConn1
  T_206686474_230000;138000;13800_Subestação_Xanxerê_Eletrosul/RConn1 -- L_206686474/LConn1
  T_206686474_230000;138000;13800_Subestação_Xanxerê_Eletrosul/RConn2 -- L_206686474/LConn2
  L_206686474/LConn3 -- T_206686474_230000;138000;13800_Subestação_Xanxerê_Eletrosul/RConn3 -- bus463/LConn1
  T_422987951__/RConn1 -- L_422987951/LConn1
  T_422987951__/RConn2 -- L_422987951/LConn2
  L_422987951/LConn3 -- T_422987951__/RConn3 -- bus464/LConn1
  T_255316432__Subestação_de_Barro_Alto/RConn1 -- L_255316432/LConn1
  T_255316432__Subestação_de_Barro_Alto/RConn2 -- L_255316432/LConn2
  L_255316432/LConn3 -- T_255316432__Subestação_de_Barro_Alto/RConn3 -- bus465/LConn1
  T_262608562__/RConn1 -- L_262608562/LConn1
  T_262608562__/RConn2 -- L_262608562/LConn2
  L_262608562/LConn3 -- T_262608562__/RConn3 -- bus466/LConn1
  T_204496577__/RConn1 -- L_204496577/LConn1
  T_204496577__/RConn2 -- L_204496577/LConn2
  L_204496577/LConn3 -- T_204496577__/RConn3 -- bus467/LConn1
  T_121809567__Livramento_2/RConn1 -- L_121809567/LConn1
  T_121809567__Livramento_2/RConn2 -- L_121809567/LConn2
  L_121809567/LConn3 -- T_121809567__Livramento_2/RConn3 -- bus468/LConn1
  T_285303568__Subestação_de_Picos/RConn1 -- L_285303568/LConn1
  T_285303568__Subestação_de_Picos/RConn2 -- L_285303568/LConn2
  L_285303568/LConn3 -- T_285303568__Subestação_de_Picos/RConn3 -- bus469/LConn1
  T_271352019__/RConn1 -- L_271352019/LConn1
  T_271352019__/RConn2 -- L_271352019/LConn2
  L_271352019/LConn3 -- T_271352019__/RConn3 -- bus470/LConn1
  T_130128162__/RConn1 -- L_130128162/LConn1
  T_130128162__/RConn2 -- L_130128162/LConn2
  L_130128162/LConn3 -- T_130128162__/RConn3 -- bus471/LConn1
  T_358443834__/RConn1 -- L_358443834/LConn1
  T_358443834__/RConn2 -- L_358443834/LConn2
  L_358443834/LConn3 -- T_358443834__/RConn3 -- bus472/LConn1
  T_240027358__Subestação_UHE_Passo_Fundo/RConn1 -- L_240027358/LConn1
  T_240027358__Subestação_UHE_Passo_Fundo/RConn2 -- L_240027358/LConn2
  L_240027358/LConn3 -- T_240027358__Subestação_UHE_Passo_Fundo/RConn3 -- bus473/LConn1
  T_251109605__Sub_estação_da_Coelba/RConn1 -- L_251109605/LConn1
  T_251109605__Sub_estação_da_Coelba/RConn2 -- L_251109605/LConn2
  L_251109605/LConn3 -- T_251109605__Sub_estação_da_Coelba/RConn3 -- bus474/LConn1
  T_307509505__Coelba/RConn1 -- L_307509505/LConn1
  T_307509505__Coelba/RConn2 -- L_307509505/LConn2
  L_307509505/LConn3 -- T_307509505__Coelba/RConn3 -- bus475/LConn1
  T_256782587__/RConn1 -- L_256782587/LConn1
  T_256782587__/RConn2 -- L_256782587/LConn2
  L_256782587/LConn3 -- T_256782587__/RConn3 -- bus476/LConn1
  T_194829553__Subestação_Figueira/RConn1 -- L_194829553/LConn1
  T_194829553__Subestação_Figueira/RConn2 -- L_194829553/LConn2
  L_194829553/LConn3 -- T_194829553__Subestação_Figueira/RConn3 -- bus477/LConn1
  T_283835652__Subestação_da_UHE_Dardanelos/RConn1 -- L_283835652/LConn1
  T_283835652__Subestação_da_UHE_Dardanelos/RConn2 -- L_283835652/LConn2
  L_283835652/LConn3 -- T_283835652__Subestação_da_UHE_Dardanelos/RConn3 -- bus478/LConn1
  T_260845425__Subestação_Juína/RConn1 -- L_260845425/LConn1
  T_260845425__Subestação_Juína/RConn2 -- L_260845425/LConn2
  L_260845425/LConn3 -- T_260845425__Subestação_Juína/RConn3 -- bus479/LConn1
  T_174067174_230000;135000_Subestação_Foz_do_Chapecó/RConn1 -- L_174067174/LConn1
  T_174067174_230000;135000_Subestação_Foz_do_Chapecó/RConn2 -- L_174067174/LConn2
  L_174067174/LConn3 -- T_174067174_230000;135000_Subestação_Foz_do_Chapecó/RConn3 -- bus480/LConn1
  T_361594711__/RConn1 -- L_361594711/LConn1
  T_361594711__/RConn2 -- L_361594711/LConn2
  L_361594711/LConn3 -- T_361594711__/RConn3 -- bus481/LConn1
  T_336967460_230000_/RConn1 -- L_336967460/LConn1
  T_336967460_230000_/RConn2 -- L_336967460/LConn2
  L_336967460/LConn3 -- T_336967460_230000_/RConn3 -- bus482/LConn1
  T_336967459_230000_/RConn1 -- L_336967459/LConn1
  T_336967459_230000_/RConn2 -- L_336967459/LConn2
  L_336967459/LConn3 -- T_336967459_230000_/RConn3 -- bus483/LConn1
  T_262932268__/RConn1 -- L_262932268/LConn1
  T_262932268__/RConn2 -- L_262932268/LConn2
  L_262932268/LConn3 -- T_262932268__/RConn3 -- bus484/LConn1
  T_221918263__Subestação_Coletora_Cerro_Chato/RConn1 -- L_221918263/LConn1
  T_221918263__Subestação_Coletora_Cerro_Chato/RConn2 -- L_221918263/LConn2
  L_221918263/LConn3 -- T_221918263__Subestação_Coletora_Cerro_Chato/RConn3 -- bus485/LConn1
  T_262608719__/RConn1 -- L_262608719/LConn1
  T_262608719__/RConn2 -- L_262608719/LConn2
  L_262608719/LConn3 -- T_262608719__/RConn3 -- bus486/LConn1
  T_216234332__/RConn1 -- L_216234332/LConn1
  T_216234332__/RConn2 -- L_216234332/LConn2
  L_216234332/LConn3 -- T_216234332__/RConn3 -- bus487/LConn1
  T_271227236__/RConn1 -- L_271227236/LConn1
  T_271227236__/RConn2 -- L_271227236/LConn2
  L_271227236/LConn3 -- T_271227236__/RConn3 -- bus488/LConn1
  T_260845424__/RConn1 -- L_260845424/LConn1
  T_260845424__/RConn2 -- L_260845424/LConn2
  L_260845424/LConn3 -- T_260845424__/RConn3 -- bus489/LConn1
  T_168946071__Subestação_Nobres/RConn1 -- L_168946071/LConn1
  T_168946071__Subestação_Nobres/RConn2 -- L_168946071/LConn2
  L_168946071/LConn3 -- T_168946071__Subestação_Nobres/RConn3 -- bus490/LConn1
  T_255316445__/RConn1 -- L_255316445/LConn1
  T_255316445__/RConn2 -- L_255316445/LConn2
  L_255316445/LConn3 -- T_255316445__/RConn3 -- bus491/LConn1
  T_171732982__Subestação_Sinop/RConn1 -- L_171732982/LConn1
  T_171732982__Subestação_Sinop/RConn2 -- L_171732982/LConn2
  L_171732982/LConn3 -- T_171732982__Subestação_Sinop/RConn3 -- bus492/LConn1
  T_259401772__Subestação_de_Corumbá_I/RConn1 -- L_259401772/LConn1
  T_259401772__Subestação_de_Corumbá_I/RConn2 -- L_259401772/LConn2
  L_259401772/LConn3 -- T_259401772__Subestação_de_Corumbá_I/RConn3 -- bus493/LConn1
  T_188413965__/RConn1 -- L_188413965/LConn1
  T_188413965__/RConn2 -- L_188413965/LConn2
